simulink model "DualStreamSSR"  (R2023a)
(part 3 of 6)

  filter15 : aieBasic/AIE Class Kernel  KernelAllAttrs=|  PortNames={'sin1'; 'sin2'; 'cin'; 'sout1'; 'sout2'}  PortSerializedTypes={'{Q2{P{Tinput_stream{1{t{Scint16}}}}}}'; '{Q2{P{Tinput_stream{1{t{Scint16}}}}}}'; '{P{Tinput_stream{1{t{Scacc48_t}}}}}'; '{Q2{P{Toutput_stream{1{t{Scint16}}}}}}'; '{Q2{P{Toutput_stream{1{t{Scint16}}}}}}'}  PortWindowSizes={0.000000000000000000e+00; 0.000000000000000000e+00; 0.000000000000000000e+00; 0.000000000000000000e+00; 0.000000000000000000e+00}  PortWindowMargins={0.000000000000000000e+00; 0.000000000000000000e+00; 0.000000000000000000e+00; 0.000000000000000000e+00; 0.000000000000000000e+00}  PortSynchronicities={'auto', 'auto', 'auto', 'auto', 'auto'}  PortSignalSizes={0.000000000000000000e+00; 0.000000000000000000e+00; 0.000000000000000000e+00; 4.000000000000000000e+00; 4.000000000000000000e+00}  ClassTemplateSpecKind=implicit  ClassTemplateParamNames={'NSamples'; 'ShiftAcc'; 'DiscardSample'; 'SwapRead'}  ClassTemplateParamKinds={'nontype'; 'nontype'; 'nontype'; 'nontype'}  ClassTemplateParamTypes={'int'; 'int'; 'bool'; 'bool'}  ClassTemplateParamValues={'512', '15', '1', '0'}  ClassCtorParamNames={'taps'}  ClassCtorParamSerializedTypes={'{R{Q1{C{Scint16}4}}}'}  ClassCtorParamValues={'[342-439i 8773+2748i 102+525i -54+21i]'}  ClassIndex=1  ClassCtorIndex=1  ClassTabVisible=on  ClassTemplateParamsVisible=on  ClassCtorDeclVisible=on  ClassCtorParamsVisible=on  FunctionTabVisible=on  FunctionDecl=|  PortAttrs={ 'input', 'sin1', 'input_stream_cint16 * restrict', '', '', '', ''; 'input', 'sin2', 'input_stream_cint16 * restrict', '', '', '', ''; 'input', 'cin', 'input_stream< cacc48_t > *', '', '', '', ''; 'output', 'sout1', 'output_stream_cint16 * restrict', '', '', '', 'OUTPUT_SIZE/2'; 'output', 'sout2', 'output_stream_cint16 * restrict', '', '', '', 'OUTPUT_SIZE/2' }  PortAttrsEnables={'off', 'off', 'off', 'off', 'off', 'off', 'off';'off', 'off', 'off', 'off', 'off', 'off', 'off';'off', 'off', 'off', 'off', 'off', 'off', 'off';'off', 'off', 'off', 'off', 'off', 'off', 'on';'off', 'off', 'off', 'off', 'off', 'off', 'on'}  SampleTime=-1  ClassDeclTypeOptions=|  ClassDecl=|  ClassTemplateParams={ 'NSamples', 'int', 'BURST_LENGTH'; 'ShiftAcc', 'int', 'SHIFT_ACC'; 'DiscardSample', 'bool', 'TRUE'; 'SwapRead', 'bool', 'FALSE' }  ClassTemplateParamsEnables={'off', 'off', 'on';'off', 'off', 'on';'off', 'off', 'on';'off', 'off', 'on'}  ClassCtorDeclTypeOptions=C[1 1]@t50@FIR_MultiKernel_cin(cint16 const ( & taps ) [ 4 ])  ClassCtorDecl=FIR_MultiKernel_cin(cint16 const ( & taps ) [ 4 ])  ClassCtorParams={ 'taps', 'cint16 const ( &) [ 4 ]', 'phi_7' }  KernelHeaderFile=FirDoubleStream.h  KernelClassName=DoubleStream::FIR_MultiKernel_cin  KernelFunction=filter  KernelSourceFile=FirDoubleStream.cpp  KernelSearchPaths={'$SRC/aie_kernels'}  PreProcOptions={}  blockJsonConstraints="{\"type\":\"constraint\",\"constraintType\":\"location_kernel\",\"sid\":\"796\",\"lhs\":{\"type\":\"location\",\"templParam\":\"kernel\",\"args\":{\"type\":\"kernel\",\"name\":\"DualStreamSSR/SSR8/filter15\",\"sid\":\"796\"}},\"rhs\":{\"type\":\"tile\",\"args\":[{\"type\":\"evaluable\",\"expr\":\"23\",\"value\":23},{\"type\":\"evaluable\",\"expr\":\"1\",\"value\":1}]},\"equality\":true}"
      KernelAllAttrs=|
      | s[12;12;9;9;19;14;21;23;24;21;12;24;26;26;26;27;28;9;21;23;23;23;24;25;14;19;19;29]@FunctionNameDeclFileNamePortNamesPortTypesPortSerializedTypesPortDirectionsPortWindowSizeEnablesPortWindowMarginEnablesPortSynchronicityEnablesPortSignalSizeEnablesFunctionDeclFunctionTemplateSpecKindFunctionTemplateParamNamesFunctionTemplateParamKindsFunctionTemplateParamTypesFunctionTemplateParamValuesFunctionTemplateParamEnablesClassDeclClassTemplateSpecKindClassTemplateParamNamesClassTemplateParamKindsClassTemplateParamTypesClassTemplateParamValuesClassTemplateParamEnablesClassCtorDeclsClassCtorParamNamesClassCtorParamTypesClassCtorParamSerializedTypes[1 1]@C[28 1]@t6@filtert42@../../../aie/aie_kernels/FirDoubleStream.hC[5 1]@t4@sin1t4@sin2t3@cint5@sout1t5@sout2C[5 1]@t30@input_stream_cint16 * restrictt30@input_stream_cint16 * restrictt26@input_stream< cacc48_t > *t31@output_stream_cint16 * restrictt31@output_stream_cint16 * restrictC[5 1]@t37@{Q2{P{Tinput_stream{1{t{Scint16}}}}}}t37@{Q2{P{Tinput_stream{1{t{Scint16}}}}}}t35@{P{Tinput_stream{1{t{Scacc48_t}}}}}t38@{Q2{P{Toutput_stream{1{t{Scint16}}}}}}t38@{Q2{P{Toutput_stream{1{t{Scint16}}}}}}C[5 1]@t5@inputt5@inputt5@inputt6@outputt6@outputC[5 1]@l0@l0@l0@l0@l0@C[5 1]@l0@l0@l0@l0@l0@C[5 1]@l0@l0@l0@l0@l0@C[5 1]@l0@l0@l0@l1@l1@t321@namespace DoubleStream {
      | template < int NSamples, int ShiftAcc, bool DiscardSample, bool SwapRead > 
      | void FIR_MultiKernel_cin::
      | filter(input_stream_cint16 * restrict sin1, input_stream_cint16 * restrict sin2, input_stream< cacc48_t > * cin, output_stream_cint16 * restrict sout1, output_stream_cint16 * restrict sout2);
      | }t4@nonee[0 1]@e[0 1]@e[0 1]@e[0 1]@e[0 1]@t128@namespace DoubleStream {
      | template < int NSamples, int ShiftAcc, bool DiscardSample, bool SwapRead > class FIR_MultiKernel_cin;
      | }t8@implicitC[4 1]@t8@NSamplest8@ShiftAcct13@DiscardSamplet8@SwapReadC[4 1]@t7@nontypet7@nontypet7@nontypet7@nontypeC[4 1]@t3@intt3@intt4@boolt4@boolC[4 1]@nnnnC[4 1]@l1@l1@l1@l1@C[1 1]@t50@FIR_MultiKernel_cin(cint16 const ( & taps ) [ 4 ])C[1 1]@C[1 1]@t4@tapsC[1 1]@C[1 1]@t23@cint16 const ( &) [ 4 ]C[1 1]@C[1 1]@t20@{R{Q1{C{Scint16}4}}}
      FunctionDecl=|
      | namespace DoubleStream {
      | template < int NSamples, int ShiftAcc, bool DiscardSample, bool SwapRead > 
      | void FIR_MultiKernel_cin::
      | filter(input_stream_cint16 * restrict sin1, input_stream_cint16 * restrict sin2, input_stream< cacc48_t > * cin, output_stream_cint16 * restrict sout1, output_stream_cint16 * restrict sout2);
      | }
      ClassDeclTypeOptions=|
      | C[1 1]@t128@namespace DoubleStream {
      | template < int NSamples, int ShiftAcc, bool DiscardSample, bool SwapRead > class FIR_MultiKernel_cin;
      | }
      ClassDecl=|
      | namespace DoubleStream {
      | template < int NSamples, int ShiftAcc, bool DiscardSample, bool SwapRead > class FIR_MultiKernel_cin;
      | }
  filter16 : aieBasic/AIE Class Kernel  KernelAllAttrs=|  PortNames={'sin1'; 'sin2'; 'cout'}  PortSerializedTypes={'{Q2{P{Tinput_stream{1{t{Scint16}}}}}}'; '{Q2{P{Tinput_stream{1{t{Scint16}}}}}}'; '{P{Toutput_stream{1{t{Scacc48_t}}}}}'}  PortWindowSizes={0.000000000000000000e+00; 0.000000000000000000e+00; 0.000000000000000000e+00}  PortWindowMargins={0.000000000000000000e+00; 0.000000000000000000e+00; 0.000000000000000000e+00}  PortSynchronicities={'auto', 'auto', 'auto'}  PortSignalSizes={0.000000000000000000e+00; 0.000000000000000000e+00; 8.000000000000000000e+00}  ClassTemplateSpecKind=implicit  ClassTemplateParamNames={'NSamples'; 'ShiftAcc'; 'DiscardSample'; 'SwapRead'}  ClassTemplateParamKinds={'nontype'; 'nontype'; 'nontype'; 'nontype'}  ClassTemplateParamTypes={'int'; 'int'; 'bool'; 'bool'}  ClassTemplateParamValues={'512', '15', '1', '0'}  ClassCtorParamNames={'taps'}  ClassCtorParamSerializedTypes={'{R{Q1{C{Scint16}4}}}'}  ClassCtorParamValues={'[146-91i 4086+5221i 237-54i -83-21i]'}  ClassIndex=1  ClassCtorIndex=1  ClassTabVisible=on  ClassTemplateParamsVisible=on  ClassCtorDeclVisible=on  ClassCtorParamsVisible=on  FunctionTabVisible=on  FunctionDecl=|  PortAttrs={ 'input', 'sin1', 'input_stream_cint16 * restrict', '', '', '', ''; 'input', 'sin2', 'input_stream_cint16 * restrict', '', '', '', ''; 'output', 'cout', 'output_stream< cacc48_t > *', '', '', '', 'OUTPUT_SIZE' }  PortAttrsEnables={'off', 'off', 'off', 'off', 'off', 'off', 'off';'off', 'off', 'off', 'off', 'off', 'off', 'off';'off', 'off', 'off', 'off', 'off', 'off', 'on'}  SampleTime=-1  ClassDeclTypeOptions=|  ClassDecl=|  ClassTemplateParams={ 'NSamples', 'int', 'BURST_LENGTH'; 'ShiftAcc', 'int', 'SHIFT_ACC'; 'DiscardSample', 'bool', 'TRUE'; 'SwapRead', 'bool', 'FALSE' }  ClassTemplateParamsEnables={'off', 'off', 'on';'off', 'off', 'on';'off', 'off', 'on';'off', 'off', 'on'}  ClassCtorDeclTypeOptions=C[1 1]@t51@FIR_MultiKernel_cout(cint16 const ( & taps ) [ 4 ])  ClassCtorDecl=FIR_MultiKernel_cout(cint16 const ( & taps ) [ 4 ])  ClassCtorParams={ 'taps', 'cint16 const ( &) [ 4 ]', 'phi_6' }  KernelHeaderFile=FirDoubleStream.h  KernelClassName=DoubleStream::FIR_MultiKernel_cout  KernelFunction=filter  KernelSourceFile=FirDoubleStream.cpp  KernelSearchPaths={'$SRC/aie_kernels'}  PreProcOptions={}  blockJsonConstraints="{\"type\":\"constraint\",\"constraintType\":\"location_kernel\",\"sid\":\"797\",\"lhs\":{\"type\":\"location\",\"templParam\":\"kernel\",\"args\":{\"type\":\"kernel\",\"name\":\"DualStreamSSR/SSR8/filter16\",\"sid\":\"797\"}},\"rhs\":{\"type\":\"tile\",\"args\":[{\"type\":\"evaluable\",\"expr\":\"23\",\"value\":23},{\"type\":\"evaluable\",\"expr\":\"2\",\"value\":2}]},\"equality\":true}"
      KernelAllAttrs=|
      | s[12;12;9;9;19;14;21;23;24;21;12;24;26;26;26;27;28;9;21;23;23;23;24;25;14;19;19;29]@FunctionNameDeclFileNamePortNamesPortTypesPortSerializedTypesPortDirectionsPortWindowSizeEnablesPortWindowMarginEnablesPortSynchronicityEnablesPortSignalSizeEnablesFunctionDeclFunctionTemplateSpecKindFunctionTemplateParamNamesFunctionTemplateParamKindsFunctionTemplateParamTypesFunctionTemplateParamValuesFunctionTemplateParamEnablesClassDeclClassTemplateSpecKindClassTemplateParamNamesClassTemplateParamKindsClassTemplateParamTypesClassTemplateParamValuesClassTemplateParamEnablesClassCtorDeclsClassCtorParamNamesClassCtorParamTypesClassCtorParamSerializedTypes[1 1]@C[28 1]@t6@filtert42@../../../aie/aie_kernels/FirDoubleStream.hC[3 1]@t4@sin1t4@sin2t4@coutC[3 1]@t30@input_stream_cint16 * restrictt30@input_stream_cint16 * restrictt27@output_stream< cacc48_t > *C[3 1]@t37@{Q2{P{Tinput_stream{1{t{Scint16}}}}}}t37@{Q2{P{Tinput_stream{1{t{Scint16}}}}}}t36@{P{Toutput_stream{1{t{Scacc48_t}}}}}C[3 1]@t5@inputt5@inputt6@outputC[3 1]@l0@l0@l0@C[3 1]@l0@l0@l0@C[3 1]@l0@l0@l0@C[3 1]@l0@l0@l1@t246@namespace DoubleStream {
      | template < int NSamples, int ShiftAcc, bool DiscardSample, bool SwapRead > 
      | void FIR_MultiKernel_cout::
      | filter(input_stream_cint16 * restrict sin1, input_stream_cint16 * restrict sin2, output_stream< cacc48_t > * cout);
      | }t4@nonee[0 1]@e[0 1]@e[0 1]@e[0 1]@e[0 1]@t129@namespace DoubleStream {
      | template < int NSamples, int ShiftAcc, bool DiscardSample, bool SwapRead > class FIR_MultiKernel_cout;
      | }t8@implicitC[4 1]@t8@NSamplest8@ShiftAcct13@DiscardSamplet8@SwapReadC[4 1]@t7@nontypet7@nontypet7@nontypet7@nontypeC[4 1]@t3@intt3@intt4@boolt4@boolC[4 1]@nnnnC[4 1]@l1@l1@l1@l1@C[1 1]@t51@FIR_MultiKernel_cout(cint16 const ( & taps ) [ 4 ])C[1 1]@C[1 1]@t4@tapsC[1 1]@C[1 1]@t23@cint16 const ( &) [ 4 ]C[1 1]@C[1 1]@t20@{R{Q1{C{Scint16}4}}}
      FunctionDecl=|
      | namespace DoubleStream {
      | template < int NSamples, int ShiftAcc, bool DiscardSample, bool SwapRead > 
      | void FIR_MultiKernel_cout::
      | filter(input_stream_cint16 * restrict sin1, input_stream_cint16 * restrict sin2, output_stream< cacc48_t > * cout);
      | }
      ClassDeclTypeOptions=|
      | C[1 1]@t129@namespace DoubleStream {
      | template < int NSamples, int ShiftAcc, bool DiscardSample, bool SwapRead > class FIR_MultiKernel_cout;
      | }
      ClassDecl=|
      | namespace DoubleStream {
      | template < int NSamples, int ShiftAcc, bool DiscardSample, bool SwapRead > class FIR_MultiKernel_cout;
      | }
  filter17 : aieBasic/AIE Class Kernel  KernelAllAttrs=|  PortNames={'sin1'; 'sin2'; 'cin'; 'cout'}  PortSerializedTypes={'{Q2{P{Tinput_stream{1{t{Scint16}}}}}}'; '{Q2{P{Tinput_stream{1{t{Scint16}}}}}}'; '{P{Tinput_stream{1{t{Scacc48_t}}}}}'; '{P{Toutput_stream{1{t{Scacc48_t}}}}}'}  PortWindowSizes={0.000000000000000000e+00; 0.000000000000000000e+00; 0.000000000000000000e+00; 0.000000000000000000e+00}  PortWindowMargins={0.000000000000000000e+00; 0.000000000000000000e+00; 0.000000000000000000e+00; 0.000000000000000000e+00}  PortSynchronicities={'auto', 'auto', 'auto', 'auto'}  PortSignalSizes={0.000000000000000000e+00; 0.000000000000000000e+00; 0.000000000000000000e+00; 8.000000000000000000e+00}  ClassTemplateSpecKind=implicit  ClassTemplateParamNames={'NSamples'; 'ShiftAcc'; 'DiscardSample'; 'SwapRead'}  ClassTemplateParamKinds={'nontype'; 'nontype'; 'nontype'; 'nontype'}  ClassTemplateParamTypes={'int'; 'int'; 'bool'; 'bool'}  ClassTemplateParamValues={'512', '15', '1', '0'}  ClassCtorParamNames={'taps'}  ClassCtorParamSerializedTypes={'{R{Q1{C{Scint16}4}}}'}  ClassCtorParamValues={'[342-439i 8773+2748i 102+525i -54+21i]'}  ClassIndex=1  ClassCtorIndex=1  ClassTabVisible=on  ClassTemplateParamsVisible=on  ClassCtorDeclVisible=on  ClassCtorParamsVisible=on  FunctionTabVisible=on  FunctionDecl=|  PortAttrs={ 'input', 'sin1', 'input_stream_cint16 * restrict', '', '', '', ''; 'input', 'sin2', 'input_stream_cint16 * restrict', '', '', '', ''; 'input', 'cin', 'input_stream< cacc48_t > *', '', '', '', ''; 'output', 'cout', 'output_stream< cacc48_t > *', '', '', '', 'OUTPUT_SIZE' }  PortAttrsEnables={'off', 'off', 'off', 'off', 'off', 'off', 'off';'off', 'off', 'off', 'off', 'off', 'off', 'off';'off', 'off', 'off', 'off', 'off', 'off', 'off';'off', 'off', 'off', 'off', 'off', 'off', 'on'}  SampleTime=-1  ClassDeclTypeOptions=|  ClassDecl=|  ClassTemplateParams={ 'NSamples', 'int', 'BURST_LENGTH'; 'ShiftAcc', 'int', 'SHIFT_ACC'; 'DiscardSample', 'bool', 'TRUE'; 'SwapRead', 'bool', 'FALSE' }  ClassTemplateParamsEnables={'off', 'off', 'on';'off', 'off', 'on';'off', 'off', 'on';'off', 'off', 'on'}  ClassCtorDeclTypeOptions=C[1 1]@t54@FIR_MultiKernel_cincout(cint16 const ( & taps ) [ 4 ])  ClassCtorDecl=FIR_MultiKernel_cincout(cint16 const ( & taps ) [ 4 ])  ClassCtorParams={ 'taps', 'cint16 const ( &) [ 4 ]', 'phi_7' }  KernelHeaderFile=FirDoubleStream.h  KernelClassName=DoubleStream::FIR_MultiKernel_cincout  KernelFunction=filter  KernelSourceFile=FirDoubleStream.cpp  KernelSearchPaths={'$SRC/aie_kernels'}  PreProcOptions={}  blockJsonConstraints="{\"type\":\"constraint\",\"constraintType\":\"location_kernel\",\"sid\":\"798\",\"lhs\":{\"type\":\"location\",\"templParam\":\"kernel\",\"args\":{\"type\":\"kernel\",\"name\":\"DualStreamSSR/SSR8/filter17\",\"sid\":\"798\"}},\"rhs\":{\"type\":\"tile\",\"args\":[{\"type\":\"evaluable\",\"expr\":\"24\",\"value\":24},{\"type\":\"evaluable\",\"expr\":\"2\",\"value\":2}]},\"equality\":true}"
      KernelAllAttrs=|
      | s[12;12;9;9;19;14;21;23;24;21;12;24;26;26;26;27;28;9;21;23;23;23;24;25;14;19;19;29]@FunctionNameDeclFileNamePortNamesPortTypesPortSerializedTypesPortDirectionsPortWindowSizeEnablesPortWindowMarginEnablesPortSynchronicityEnablesPortSignalSizeEnablesFunctionDeclFunctionTemplateSpecKindFunctionTemplateParamNamesFunctionTemplateParamKindsFunctionTemplateParamTypesFunctionTemplateParamValuesFunctionTemplateParamEnablesClassDeclClassTemplateSpecKindClassTemplateParamNamesClassTemplateParamKindsClassTemplateParamTypesClassTemplateParamValuesClassTemplateParamEnablesClassCtorDeclsClassCtorParamNamesClassCtorParamTypesClassCtorParamSerializedTypes[1 1]@C[28 1]@t6@filtert42@../../../aie/aie_kernels/FirDoubleStream.hC[4 1]@t4@sin1t4@sin2t3@cint4@coutC[4 1]@t30@input_stream_cint16 * restrictt30@input_stream_cint16 * restrictt26@input_stream< cacc48_t > *t27@output_stream< cacc48_t > *C[4 1]@t37@{Q2{P{Tinput_stream{1{t{Scint16}}}}}}t37@{Q2{P{Tinput_stream{1{t{Scint16}}}}}}t35@{P{Tinput_stream{1{t{Scacc48_t}}}}}t36@{P{Toutput_stream{1{t{Scacc48_t}}}}}C[4 1]@t5@inputt5@inputt5@inputt6@outputC[4 1]@l0@l0@l0@l0@C[4 1]@l0@l0@l0@l0@C[4 1]@l0@l0@l0@l0@C[4 1]@l0@l0@l0@l1@t281@namespace DoubleStream {
      | template < int NSamples, int ShiftAcc, bool DiscardSample, bool SwapRead > 
      | void FIR_MultiKernel_cincout::
      | filter(input_stream_cint16 * restrict sin1, input_stream_cint16 * restrict sin2, input_stream< cacc48_t > * cin, output_stream< cacc48_t > * cout);
      | }t4@nonee[0 1]@e[0 1]@e[0 1]@e[0 1]@e[0 1]@t132@namespace DoubleStream {
      | template < int NSamples, int ShiftAcc, bool DiscardSample, bool SwapRead > class FIR_MultiKernel_cincout;
      | }t8@implicitC[4 1]@t8@NSamplest8@ShiftAcct13@DiscardSamplet8@SwapReadC[4 1]@t7@nontypet7@nontypet7@nontypet7@nontypeC[4 1]@t3@intt3@intt4@boolt4@boolC[4 1]@nnnnC[4 1]@l1@l1@l1@l1@C[1 1]@t54@FIR_MultiKernel_cincout(cint16 const ( & taps ) [ 4 ])C[1 1]@C[1 1]@t4@tapsC[1 1]@C[1 1]@t23@cint16 const ( &) [ 4 ]C[1 1]@C[1 1]@t20@{R{Q1{C{Scint16}4}}}
      FunctionDecl=|
      | namespace DoubleStream {
      | template < int NSamples, int ShiftAcc, bool DiscardSample, bool SwapRead > 
      | void FIR_MultiKernel_cincout::
      | filter(input_stream_cint16 * restrict sin1, input_stream_cint16 * restrict sin2, input_stream< cacc48_t > * cin, output_stream< cacc48_t > * cout);
      | }
      ClassDeclTypeOptions=|
      | C[1 1]@t132@namespace DoubleStream {
      | template < int NSamples, int ShiftAcc, bool DiscardSample, bool SwapRead > class FIR_MultiKernel_cincout;
      | }
      ClassDecl=|
      | namespace DoubleStream {
      | template < int NSamples, int ShiftAcc, bool DiscardSample, bool SwapRead > class FIR_MultiKernel_cincout;
      | }
  filter18 : aieBasic/AIE Class Kernel  KernelAllAttrs=|  PortNames={'sin1'; 'sin2'; 'cin'; 'cout'}  PortSerializedTypes={'{Q2{P{Tinput_stream{1{t{Scint16}}}}}}'; '{Q2{P{Tinput_stream{1{t{Scint16}}}}}}'; '{P{Tinput_stream{1{t{Scacc48_t}}}}}'; '{P{Toutput_stream{1{t{Scacc48_t}}}}}'}  PortWindowSizes={0.000000000000000000e+00; 0.000000000000000000e+00; 0.000000000000000000e+00; 0.000000000000000000e+00}  PortWindowMargins={0.000000000000000000e+00; 0.000000000000000000e+00; 0.000000000000000000e+00; 0.000000000000000000e+00}  PortSynchronicities={'auto', 'auto', 'auto', 'auto'}  PortSignalSizes={0.000000000000000000e+00; 0.000000000000000000e+00; 0.000000000000000000e+00; 8.000000000000000000e+00}  ClassTemplateSpecKind=implicit  ClassTemplateParamNames={'NSamples'; 'ShiftAcc'; 'DiscardSample'; 'SwapRead'}  ClassTemplateParamKinds={'nontype'; 'nontype'; 'nontype'; 'nontype'}  ClassTemplateParamTypes={'int'; 'int'; 'bool'; 'bool'}  ClassTemplateParamValues={'512', '15', '1', '0'}  ClassCtorParamNames={'taps'}  ClassCtorParamSerializedTypes={'{R{Q1{C{Scint16}4}}}'}  ClassCtorParamValues={'[342-439i 8773+2748i 102+525i -54+21i]'}  ClassIndex=1  ClassCtorIndex=1  ClassTabVisible=on  ClassTemplateParamsVisible=on  ClassCtorDeclVisible=on  ClassCtorParamsVisible=on  FunctionTabVisible=on  FunctionDecl=|  PortAttrs={ 'input', 'sin1', 'input_stream_cint16 * restrict', '', '', '', ''; 'input', 'sin2', 'input_stream_cint16 * restrict', '', '', '', ''; 'input', 'cin', 'input_stream< cacc48_t > *', '', '', '', ''; 'output', 'cout', 'output_stream< cacc48_t > *', '', '', '', 'OUTPUT_SIZE' }  PortAttrsEnables={'off', 'off', 'off', 'off', 'off', 'off', 'off';'off', 'off', 'off', 'off', 'off', 'off', 'off';'off', 'off', 'off', 'off', 'off', 'off', 'off';'off', 'off', 'off', 'off', 'off', 'off', 'on'}  SampleTime=-1  ClassDeclTypeOptions=|  ClassDecl=|  ClassTemplateParams={ 'NSamples', 'int', 'BURST_LENGTH'; 'ShiftAcc', 'int', 'SHIFT_ACC'; 'DiscardSample', 'bool', 'TRUE'; 'SwapRead', 'bool', 'FALSE' }  ClassTemplateParamsEnables={'off', 'off', 'on';'off', 'off', 'on';'off', 'off', 'on';'off', 'off', 'on'}  ClassCtorDeclTypeOptions=C[1 1]@t54@FIR_MultiKernel_cincout(cint16 const ( & taps ) [ 4 ])  ClassCtorDecl=FIR_MultiKernel_cincout(cint16 const ( & taps ) [ 4 ])  ClassCtorParams={ 'taps', 'cint16 const ( &) [ 4 ]', 'phi_7' }  KernelHeaderFile=FirDoubleStream.h  KernelClassName=DoubleStream::FIR_MultiKernel_cincout  KernelFunction=filter  KernelSourceFile=FirDoubleStream.cpp  KernelSearchPaths={'$SRC/aie_kernels'}  PreProcOptions={}  blockJsonConstraints="{\"type\":\"constraint\",\"constraintType\":\"location_kernel\",\"sid\":\"799\",\"lhs\":{\"type\":\"location\",\"templParam\":\"kernel\",\"args\":{\"type\":\"kernel\",\"name\":\"DualStreamSSR/SSR8/filter18\",\"sid\":\"799\"}},\"rhs\":{\"type\":\"tile\",\"args\":[{\"type\":\"evaluable\",\"expr\":\"25\",\"value\":25},{\"type\":\"evaluable\",\"expr\":\"3\",\"value\":3}]},\"equality\":true}"
      KernelAllAttrs=|
      | s[12;12;9;9;19;14;21;23;24;21;12;24;26;26;26;27;28;9;21;23;23;23;24;25;14;19;19;29]@FunctionNameDeclFileNamePortNamesPortTypesPortSerializedTypesPortDirectionsPortWindowSizeEnablesPortWindowMarginEnablesPortSynchronicityEnablesPortSignalSizeEnablesFunctionDeclFunctionTemplateSpecKindFunctionTemplateParamNamesFunctionTemplateParamKindsFunctionTemplateParamTypesFunctionTemplateParamValuesFunctionTemplateParamEnablesClassDeclClassTemplateSpecKindClassTemplateParamNamesClassTemplateParamKindsClassTemplateParamTypesClassTemplateParamValuesClassTemplateParamEnablesClassCtorDeclsClassCtorParamNamesClassCtorParamTypesClassCtorParamSerializedTypes[1 1]@C[28 1]@t6@filtert42@../../../aie/aie_kernels/FirDoubleStream.hC[4 1]@t4@sin1t4@sin2t3@cint4@coutC[4 1]@t30@input_stream_cint16 * restrictt30@input_stream_cint16 * restrictt26@input_stream< cacc48_t > *t27@output_stream< cacc48_t > *C[4 1]@t37@{Q2{P{Tinput_stream{1{t{Scint16}}}}}}t37@{Q2{P{Tinput_stream{1{t{Scint16}}}}}}t35@{P{Tinput_stream{1{t{Scacc48_t}}}}}t36@{P{Toutput_stream{1{t{Scacc48_t}}}}}C[4 1]@t5@inputt5@inputt5@inputt6@outputC[4 1]@l0@l0@l0@l0@C[4 1]@l0@l0@l0@l0@C[4 1]@l0@l0@l0@l0@C[4 1]@l0@l0@l0@l1@t281@namespace DoubleStream {
      | template < int NSamples, int ShiftAcc, bool DiscardSample, bool SwapRead > 
      | void FIR_MultiKernel_cincout::
      | filter(input_stream_cint16 * restrict sin1, input_stream_cint16 * restrict sin2, input_stream< cacc48_t > * cin, output_stream< cacc48_t > * cout);
      | }t4@nonee[0 1]@e[0 1]@e[0 1]@e[0 1]@e[0 1]@t132@namespace DoubleStream {
      | template < int NSamples, int ShiftAcc, bool DiscardSample, bool SwapRead > class FIR_MultiKernel_cincout;
      | }t8@implicitC[4 1]@t8@NSamplest8@ShiftAcct13@DiscardSamplet8@SwapReadC[4 1]@t7@nontypet7@nontypet7@nontypet7@nontypeC[4 1]@t3@intt3@intt4@boolt4@boolC[4 1]@nnnnC[4 1]@l1@l1@l1@l1@C[1 1]@t54@FIR_MultiKernel_cincout(cint16 const ( & taps ) [ 4 ])C[1 1]@C[1 1]@t4@tapsC[1 1]@C[1 1]@t23@cint16 const ( &) [ 4 ]C[1 1]@C[1 1]@t20@{R{Q1{C{Scint16}4}}}
      FunctionDecl=|
      | namespace DoubleStream {
      | template < int NSamples, int ShiftAcc, bool DiscardSample, bool SwapRead > 
      | void FIR_MultiKernel_cincout::
      | filter(input_stream_cint16 * restrict sin1, input_stream_cint16 * restrict sin2, input_stream< cacc48_t > * cin, output_stream< cacc48_t > * cout);
      | }
      ClassDeclTypeOptions=|
      | C[1 1]@t132@namespace DoubleStream {
      | template < int NSamples, int ShiftAcc, bool DiscardSample, bool SwapRead > class FIR_MultiKernel_cincout;
      | }
      ClassDecl=|
      | namespace DoubleStream {
      | template < int NSamples, int ShiftAcc, bool DiscardSample, bool SwapRead > class FIR_MultiKernel_cincout;
      | }
  filter19 : aieBasic/AIE Class Kernel  KernelAllAttrs=|  PortNames={'sin1'; 'sin2'; 'cin'; 'cout'}  PortSerializedTypes={'{Q2{P{Tinput_stream{1{t{Scint16}}}}}}'; '{Q2{P{Tinput_stream{1{t{Scint16}}}}}}'; '{P{Tinput_stream{1{t{Scacc48_t}}}}}'; '{P{Toutput_stream{1{t{Scacc48_t}}}}}'}  PortWindowSizes={0.000000000000000000e+00; 0.000000000000000000e+00; 0.000000000000000000e+00; 0.000000000000000000e+00}  PortWindowMargins={0.000000000000000000e+00; 0.000000000000000000e+00; 0.000000000000000000e+00; 0.000000000000000000e+00}  PortSynchronicities={'auto', 'auto', 'auto', 'auto'}  PortSignalSizes={0.000000000000000000e+00; 0.000000000000000000e+00; 0.000000000000000000e+00; 8.000000000000000000e+00}  ClassTemplateSpecKind=implicit  ClassTemplateParamNames={'NSamples'; 'ShiftAcc'; 'DiscardSample'; 'SwapRead'}  ClassTemplateParamKinds={'nontype'; 'nontype'; 'nontype'; 'nontype'}  ClassTemplateParamTypes={'int'; 'int'; 'bool'; 'bool'}  ClassTemplateParamValues={'512', '15', '0', '0'}  ClassCtorParamNames={'taps'}  ClassCtorParamSerializedTypes={'{R{Q1{C{Scint16}4}}}'}  ClassCtorParamValues={'[-54-21i 102-525i 8773-2748i 342+439i]'}  ClassIndex=1  ClassCtorIndex=1  ClassTabVisible=on  ClassTemplateParamsVisible=on  ClassCtorDeclVisible=on  ClassCtorParamsVisible=on  FunctionTabVisible=on  FunctionDecl=|  PortAttrs={ 'input', 'sin1', 'input_stream_cint16 * restrict', '', '', '', ''; 'input', 'sin2', 'input_stream_cint16 * restrict', '', '', '', ''; 'input', 'cin', 'input_stream< cacc48_t > *', '', '', '', ''; 'output', 'cout', 'output_stream< cacc48_t > *', '', '', '', 'OUTPUT_SIZE' }  PortAttrsEnables={'off', 'off', 'off', 'off', 'off', 'off', 'off';'off', 'off', 'off', 'off', 'off', 'off', 'off';'off', 'off', 'off', 'off', 'off', 'off', 'off';'off', 'off', 'off', 'off', 'off', 'off', 'on'}  SampleTime=-1  ClassDeclTypeOptions=|  ClassDecl=|  ClassTemplateParams={ 'NSamples', 'int', 'BURST_LENGTH'; 'ShiftAcc', 'int', 'SHIFT_ACC'; 'DiscardSample', 'bool', 'FALSE'; 'SwapRead', 'bool', 'FALSE' }  ClassTemplateParamsEnables={'off', 'off', 'on';'off', 'off', 'on';'off', 'off', 'on';'off', 'off', 'on'}  ClassCtorDeclTypeOptions=C[1 1]@t54@FIR_MultiKernel_cincout(cint16 const ( & taps ) [ 4 ])  ClassCtorDecl=FIR_MultiKernel_cincout(cint16 const ( & taps ) [ 4 ])  ClassCtorParams={ 'taps', 'cint16 const ( &) [ 4 ]', 'phi_0' }  KernelHeaderFile=FirDoubleStream.h  KernelClassName=DoubleStream::FIR_MultiKernel_cincout  KernelFunction=filter  KernelSourceFile=FirDoubleStream.cpp  KernelSearchPaths={'$SRC/aie_kernels'}  PreProcOptions={}  blockJsonConstraints="{\"type\":\"constraint\",\"constraintType\":\"location_kernel\",\"sid\":\"800\",\"lhs\":{\"type\":\"location\",\"templParam\":\"kernel\",\"args\":{\"type\":\"kernel\",\"name\":\"DualStreamSSR/SSR8/filter19\",\"sid\":\"800\"}},\"rhs\":{\"type\":\"tile\",\"args\":[{\"type\":\"evaluable\",\"expr\":\"26\",\"value\":26},{\"type\":\"evaluable\",\"expr\":\"3\",\"value\":3}]},\"equality\":true}"
      KernelAllAttrs=|
      | s[12;12;9;9;19;14;21;23;24;21;12;24;26;26;26;27;28;9;21;23;23;23;24;25;14;19;19;29]@FunctionNameDeclFileNamePortNamesPortTypesPortSerializedTypesPortDirectionsPortWindowSizeEnablesPortWindowMarginEnablesPortSynchronicityEnablesPortSignalSizeEnablesFunctionDeclFunctionTemplateSpecKindFunctionTemplateParamNamesFunctionTemplateParamKindsFunctionTemplateParamTypesFunctionTemplateParamValuesFunctionTemplateParamEnablesClassDeclClassTemplateSpecKindClassTemplateParamNamesClassTemplateParamKindsClassTemplateParamTypesClassTemplateParamValuesClassTemplateParamEnablesClassCtorDeclsClassCtorParamNamesClassCtorParamTypesClassCtorParamSerializedTypes[1 1]@C[28 1]@t6@filtert42@../../../aie/aie_kernels/FirDoubleStream.hC[4 1]@t4@sin1t4@sin2t3@cint4@coutC[4 1]@t30@input_stream_cint16 * restrictt30@input_stream_cint16 * restrictt26@input_stream< cacc48_t > *t27@output_stream< cacc48_t > *C[4 1]@t37@{Q2{P{Tinput_stream{1{t{Scint16}}}}}}t37@{Q2{P{Tinput_stream{1{t{Scint16}}}}}}t35@{P{Tinput_stream{1{t{Scacc48_t}}}}}t36@{P{Toutput_stream{1{t{Scacc48_t}}}}}C[4 1]@t5@inputt5@inputt5@inputt6@outputC[4 1]@l0@l0@l0@l0@C[4 1]@l0@l0@l0@l0@C[4 1]@l0@l0@l0@l0@C[4 1]@l0@l0@l0@l1@t281@namespace DoubleStream {
      | template < int NSamples, int ShiftAcc, bool DiscardSample, bool SwapRead > 
      | void FIR_MultiKernel_cincout::
      | filter(input_stream_cint16 * restrict sin1, input_stream_cint16 * restrict sin2, input_stream< cacc48_t > * cin, output_stream< cacc48_t > * cout);
      | }t4@nonee[0 1]@e[0 1]@e[0 1]@e[0 1]@e[0 1]@t132@namespace DoubleStream {
      | template < int NSamples, int ShiftAcc, bool DiscardSample, bool SwapRead > class FIR_MultiKernel_cincout;
      | }t8@implicitC[4 1]@t8@NSamplest8@ShiftAcct13@DiscardSamplet8@SwapReadC[4 1]@t7@nontypet7@nontypet7@nontypet7@nontypeC[4 1]@t3@intt3@intt4@boolt4@boolC[4 1]@nnnnC[4 1]@l1@l1@l1@l1@C[1 1]@t54@FIR_MultiKernel_cincout(cint16 const ( & taps ) [ 4 ])C[1 1]@C[1 1]@t4@tapsC[1 1]@C[1 1]@t23@cint16 const ( &) [ 4 ]C[1 1]@C[1 1]@t20@{R{Q1{C{Scint16}4}}}
      FunctionDecl=|
      | namespace DoubleStream {
      | template < int NSamples, int ShiftAcc, bool DiscardSample, bool SwapRead > 
      | void FIR_MultiKernel_cincout::
      | filter(input_stream_cint16 * restrict sin1, input_stream_cint16 * restrict sin2, input_stream< cacc48_t > * cin, output_stream< cacc48_t > * cout);
      | }
      ClassDeclTypeOptions=|
      | C[1 1]@t132@namespace DoubleStream {
      | template < int NSamples, int ShiftAcc, bool DiscardSample, bool SwapRead > class FIR_MultiKernel_cincout;
      | }
      ClassDecl=|
      | namespace DoubleStream {
      | template < int NSamples, int ShiftAcc, bool DiscardSample, bool SwapRead > class FIR_MultiKernel_cincout;
      | }
  filter2 : aieBasic/AIE Class Kernel  KernelAllAttrs=|  PortNames={'sin1'; 'sin2'; 'cin'; 'cout'}  PortSerializedTypes={'{Q2{P{Tinput_stream{1{t{Scint16}}}}}}'; '{Q2{P{Tinput_stream{1{t{Scint16}}}}}}'; '{P{Tinput_stream{1{t{Scacc48_t}}}}}'; '{P{Toutput_stream{1{t{Scacc48_t}}}}}'}  PortWindowSizes={0.000000000000000000e+00; 0.000000000000000000e+00; 0.000000000000000000e+00; 0.000000000000000000e+00}  PortWindowMargins={0.000000000000000000e+00; 0.000000000000000000e+00; 0.000000000000000000e+00; 0.000000000000000000e+00}  PortSynchronicities={'auto', 'auto', 'auto', 'auto'}  PortSignalSizes={0.000000000000000000e+00; 0.000000000000000000e+00; 0.000000000000000000e+00; 8.000000000000000000e+00}  ClassTemplateSpecKind=implicit  ClassTemplateParamNames={'NSamples'; 'ShiftAcc'; 'DiscardSample'; 'SwapRead'}  ClassTemplateParamKinds={'nontype'; 'nontype'; 'nontype'; 'nontype'}  ClassTemplateParamTypes={'int'; 'int'; 'bool'; 'bool'}  ClassTemplateParamValues={'512', '15', '0', '0'}  ClassCtorParamNames={'taps'}  ClassCtorParamSerializedTypes={'{R{Q1{C{Scint16}4}}}'}  ClassCtorParamValues={'[-21+26i 1183+239i 248-2878i -160+111i]'}  ClassIndex=1  ClassCtorIndex=1  ClassTabVisible=on  ClassTemplateParamsVisible=on  ClassCtorDeclVisible=on  ClassCtorParamsVisible=on  FunctionTabVisible=on  FunctionDecl=|  PortAttrs={ 'input', 'sin1', 'input_stream_cint16 * restrict', '', '', '', ''; 'input', 'sin2', 'input_stream_cint16 * restrict', '', '', '', ''; 'input', 'cin', 'input_stream< cacc48_t > *', '', '', '', ''; 'output', 'cout', 'output_stream< cacc48_t > *', '', '', '', 'OUTPUT_SIZE' }  PortAttrsEnables={'off', 'off', 'off', 'off', 'off', 'off', 'off';'off', 'off', 'off', 'off', 'off', 'off', 'off';'off', 'off', 'off', 'off', 'off', 'off', 'off';'off', 'off', 'off', 'off', 'off', 'off', 'on'}  SampleTime=-1  ClassDeclTypeOptions=|  ClassDecl=|  ClassTemplateParams={ 'NSamples', 'int', 'BURST_LENGTH'; 'ShiftAcc', 'int', 'SHIFT_ACC'; 'DiscardSample', 'bool', 'FALSE'; 'SwapRead', 'bool', 'FALSE' }  ClassTemplateParamsEnables={'off', 'off', 'on';'off', 'off', 'on';'off', 'off', 'on';'off', 'off', 'on'}  ClassCtorDeclTypeOptions=C[1 1]@t54@FIR_MultiKernel_cincout(cint16 const ( & taps ) [ 4 ])  ClassCtorDecl=FIR_MultiKernel_cincout(cint16 const ( & taps ) [ 4 ])  ClassCtorParams={ 'taps', 'cint16 const ( &) [ 4 ]', 'phi_2' }  KernelHeaderFile=FirDoubleStream.h  KernelClassName=DoubleStream::FIR_MultiKernel_cincout  KernelFunction=filter  KernelSourceFile=FirDoubleStream.cpp  KernelSearchPaths={'$SRC/aie_kernels'}  PreProcOptions={}  blockJsonConstraints="{\"type\":\"constraint\",\"constraintType\":\"location_kernel\",\"sid\":\"801\",\"lhs\":{\"type\":\"location\",\"templParam\":\"kernel\",\"args\":{\"type\":\"kernel\",\"name\":\"DualStreamSSR/SSR8/filter2\",\"sid\":\"801\"}},\"rhs\":{\"type\":\"tile\",\"args\":[{\"type\":\"evaluable\",\"expr\":\"25\",\"value\":25},{\"type\":\"evaluable\",\"expr\":\"0\",\"value\":0}]},\"equality\":true}"
      KernelAllAttrs=|
      | s[12;12;9;9;19;14;21;23;24;21;12;24;26;26;26;27;28;9;21;23;23;23;24;25;14;19;19;29]@FunctionNameDeclFileNamePortNamesPortTypesPortSerializedTypesPortDirectionsPortWindowSizeEnablesPortWindowMarginEnablesPortSynchronicityEnablesPortSignalSizeEnablesFunctionDeclFunctionTemplateSpecKindFunctionTemplateParamNamesFunctionTemplateParamKindsFunctionTemplateParamTypesFunctionTemplateParamValuesFunctionTemplateParamEnablesClassDeclClassTemplateSpecKindClassTemplateParamNamesClassTemplateParamKindsClassTemplateParamTypesClassTemplateParamValuesClassTemplateParamEnablesClassCtorDeclsClassCtorParamNamesClassCtorParamTypesClassCtorParamSerializedTypes[1 1]@C[28 1]@t6@filtert42@../../../aie/aie_kernels/FirDoubleStream.hC[4 1]@t4@sin1t4@sin2t3@cint4@coutC[4 1]@t30@input_stream_cint16 * restrictt30@input_stream_cint16 * restrictt26@input_stream< cacc48_t > *t27@output_stream< cacc48_t > *C[4 1]@t37@{Q2{P{Tinput_stream{1{t{Scint16}}}}}}t37@{Q2{P{Tinput_stream{1{t{Scint16}}}}}}t35@{P{Tinput_stream{1{t{Scacc48_t}}}}}t36@{P{Toutput_stream{1{t{Scacc48_t}}}}}C[4 1]@t5@inputt5@inputt5@inputt6@outputC[4 1]@l0@l0@l0@l0@C[4 1]@l0@l0@l0@l0@C[4 1]@l0@l0@l0@l0@C[4 1]@l0@l0@l0@l1@t281@namespace DoubleStream {
      | template < int NSamples, int ShiftAcc, bool DiscardSample, bool SwapRead > 
      | void FIR_MultiKernel_cincout::
      | filter(input_stream_cint16 * restrict sin1, input_stream_cint16 * restrict sin2, input_stream< cacc48_t > * cin, output_stream< cacc48_t > * cout);
      | }t4@nonee[0 1]@e[0 1]@e[0 1]@e[0 1]@e[0 1]@t132@namespace DoubleStream {
      | template < int NSamples, int ShiftAcc, bool DiscardSample, bool SwapRead > class FIR_MultiKernel_cincout;
      | }t8@implicitC[4 1]@t8@NSamplest8@ShiftAcct13@DiscardSamplet8@SwapReadC[4 1]@t7@nontypet7@nontypet7@nontypet7@nontypeC[4 1]@t3@intt3@intt4@boolt4@boolC[4 1]@nnnnC[4 1]@l1@l1@l1@l1@C[1 1]@t54@FIR_MultiKernel_cincout(cint16 const ( & taps ) [ 4 ])C[1 1]@C[1 1]@t4@tapsC[1 1]@C[1 1]@t23@cint16 const ( &) [ 4 ]C[1 1]@C[1 1]@t20@{R{Q1{C{Scint16}4}}}
      FunctionDecl=|
      | namespace DoubleStream {
      | template < int NSamples, int ShiftAcc, bool DiscardSample, bool SwapRead > 
      | void FIR_MultiKernel_cincout::
      | filter(input_stream_cint16 * restrict sin1, input_stream_cint16 * restrict sin2, input_stream< cacc48_t > * cin, output_stream< cacc48_t > * cout);
      | }
      ClassDeclTypeOptions=|
      | C[1 1]@t132@namespace DoubleStream {
      | template < int NSamples, int ShiftAcc, bool DiscardSample, bool SwapRead > class FIR_MultiKernel_cincout;
      | }
      ClassDecl=|
      | namespace DoubleStream {
      | template < int NSamples, int ShiftAcc, bool DiscardSample, bool SwapRead > class FIR_MultiKernel_cincout;
      | }
  filter20 : aieBasic/AIE Class Kernel  KernelAllAttrs=|  PortNames={'sin1'; 'sin2'; 'cin'; 'cout'}  PortSerializedTypes={'{Q2{P{Tinput_stream{1{t{Scint16}}}}}}'; '{Q2{P{Tinput_stream{1{t{Scint16}}}}}}'; '{P{Tinput_stream{1{t{Scacc48_t}}}}}'; '{P{Toutput_stream{1{t{Scacc48_t}}}}}'}  PortWindowSizes={0.000000000000000000e+00; 0.000000000000000000e+00; 0.000000000000000000e+00; 0.000000000000000000e+00}  PortWindowMargins={0.000000000000000000e+00; 0.000000000000000000e+00; 0.000000000000000000e+00; 0.000000000000000000e+00}  PortSynchronicities={'auto', 'auto', 'auto', 'auto'}  PortSignalSizes={0.000000000000000000e+00; 0.000000000000000000e+00; 0.000000000000000000e+00; 8.000000000000000000e+00}  ClassTemplateSpecKind=implicit  ClassTemplateParamNames={'NSamples'; 'ShiftAcc'; 'DiscardSample'; 'SwapRead'}  ClassTemplateParamKinds={'nontype'; 'nontype'; 'nontype'; 'nontype'}  ClassTemplateParamTypes={'int'; 'int'; 'bool'; 'bool'}  ClassTemplateParamValues={'512', '15', '0', '0'}  ClassCtorParamNames={'taps'}  ClassCtorParamSerializedTypes={'{R{Q1{C{Scint16}4}}}'}  ClassCtorParamValues={'[-83+21i 237+54i 4086-5221i 146+91i]'}  ClassIndex=1  ClassCtorIndex=1  ClassTabVisible=on  ClassTemplateParamsVisible=on  ClassCtorDeclVisible=on  ClassCtorParamsVisible=on  FunctionTabVisible=on  FunctionDecl=|  PortAttrs={ 'input', 'sin1', 'input_stream_cint16 * restrict', '', '', '', ''; 'input', 'sin2', 'input_stream_cint16 * restrict', '', '', '', ''; 'input', 'cin', 'input_stream< cacc48_t > *', '', '', '', ''; 'output', 'cout', 'output_stream< cacc48_t > *', '', '', '', 'OUTPUT_SIZE' }  PortAttrsEnables={'off', 'off', 'off', 'off', 'off', 'off', 'off';'off', 'off', 'off', 'off', 'off', 'off', 'off';'off', 'off', 'off', 'off', 'off', 'off', 'off';'off', 'off', 'off', 'off', 'off', 'off', 'on'}  SampleTime=-1  ClassDeclTypeOptions=|  ClassDecl=|  ClassTemplateParams={ 'NSamples', 'int', 'BURST_LENGTH'; 'ShiftAcc', 'int', 'SHIFT_ACC'; 'DiscardSample', 'bool', 'FALSE'; 'SwapRead', 'bool', 'FALSE' }  ClassTemplateParamsEnables={'off', 'off', 'on';'off', 'off', 'on';'off', 'off', 'on';'off', 'off', 'on'}  ClassCtorDeclTypeOptions=C[1 1]@t54@FIR_MultiKernel_cincout(cint16 const ( & taps ) [ 4 ])  ClassCtorDecl=FIR_MultiKernel_cincout(cint16 const ( & taps ) [ 4 ])  ClassCtorParams={ 'taps', 'cint16 const ( &) [ 4 ]', 'phi_1' }  KernelHeaderFile=FirDoubleStream.h  KernelClassName=DoubleStream::FIR_MultiKernel_cincout  KernelFunction=filter  KernelSourceFile=FirDoubleStream.cpp  KernelSearchPaths={'$SRC/aie_kernels'}  PreProcOptions={}  blockJsonConstraints="{\"type\":\"constraint\",\"constraintType\":\"location_kernel\",\"sid\":\"802\",\"lhs\":{\"type\":\"location\",\"templParam\":\"kernel\",\"args\":{\"type\":\"kernel\",\"name\":\"DualStreamSSR/SSR8/filter20\",\"sid\":\"802\"}},\"rhs\":{\"type\":\"tile\",\"args\":[{\"type\":\"evaluable\",\"expr\":\"27\",\"value\":27},{\"type\":\"evaluable\",\"expr\":\"3\",\"value\":3}]},\"equality\":true}"
      KernelAllAttrs=|
      | s[12;12;9;9;19;14;21;23;24;21;12;24;26;26;26;27;28;9;21;23;23;23;24;25;14;19;19;29]@FunctionNameDeclFileNamePortNamesPortTypesPortSerializedTypesPortDirectionsPortWindowSizeEnablesPortWindowMarginEnablesPortSynchronicityEnablesPortSignalSizeEnablesFunctionDeclFunctionTemplateSpecKindFunctionTemplateParamNamesFunctionTemplateParamKindsFunctionTemplateParamTypesFunctionTemplateParamValuesFunctionTemplateParamEnablesClassDeclClassTemplateSpecKindClassTemplateParamNamesClassTemplateParamKindsClassTemplateParamTypesClassTemplateParamValuesClassTemplateParamEnablesClassCtorDeclsClassCtorParamNamesClassCtorParamTypesClassCtorParamSerializedTypes[1 1]@C[28 1]@t6@filtert42@../../../aie/aie_kernels/FirDoubleStream.hC[4 1]@t4@sin1t4@sin2t3@cint4@coutC[4 1]@t30@input_stream_cint16 * restrictt30@input_stream_cint16 * restrictt26@input_stream< cacc48_t > *t27@output_stream< cacc48_t > *C[4 1]@t37@{Q2{P{Tinput_stream{1{t{Scint16}}}}}}t37@{Q2{P{Tinput_stream{1{t{Scint16}}}}}}t35@{P{Tinput_stream{1{t{Scacc48_t}}}}}t36@{P{Toutput_stream{1{t{Scacc48_t}}}}}C[4 1]@t5@inputt5@inputt5@inputt6@outputC[4 1]@l0@l0@l0@l0@C[4 1]@l0@l0@l0@l0@C[4 1]@l0@l0@l0@l0@C[4 1]@l0@l0@l0@l1@t281@namespace DoubleStream {
      | template < int NSamples, int ShiftAcc, bool DiscardSample, bool SwapRead > 
      | void FIR_MultiKernel_cincout::
      | filter(input_stream_cint16 * restrict sin1, input_stream_cint16 * restrict sin2, input_stream< cacc48_t > * cin, output_stream< cacc48_t > * cout);
      | }t4@nonee[0 1]@e[0 1]@e[0 1]@e[0 1]@e[0 1]@t132@namespace DoubleStream {
      | template < int NSamples, int ShiftAcc, bool DiscardSample, bool SwapRead > class FIR_MultiKernel_cincout;
      | }t8@implicitC[4 1]@t8@NSamplest8@ShiftAcct13@DiscardSamplet8@SwapReadC[4 1]@t7@nontypet7@nontypet7@nontypet7@nontypeC[4 1]@t3@intt3@intt4@boolt4@boolC[4 1]@nnnnC[4 1]@l1@l1@l1@l1@C[1 1]@t54@FIR_MultiKernel_cincout(cint16 const ( & taps ) [ 4 ])C[1 1]@C[1 1]@t4@tapsC[1 1]@C[1 1]@t23@cint16 const ( &) [ 4 ]C[1 1]@C[1 1]@t20@{R{Q1{C{Scint16}4}}}
      FunctionDecl=|
      | namespace DoubleStream {
      | template < int NSamples, int ShiftAcc, bool DiscardSample, bool SwapRead > 
      | void FIR_MultiKernel_cincout::
      | filter(input_stream_cint16 * restrict sin1, input_stream_cint16 * restrict sin2, input_stream< cacc48_t > * cin, output_stream< cacc48_t > * cout);
      | }
      ClassDeclTypeOptions=|
      | C[1 1]@t132@namespace DoubleStream {
      | template < int NSamples, int ShiftAcc, bool DiscardSample, bool SwapRead > class FIR_MultiKernel_cincout;
      | }
      ClassDecl=|
      | namespace DoubleStream {
      | template < int NSamples, int ShiftAcc, bool DiscardSample, bool SwapRead > class FIR_MultiKernel_cincout;
      | }
  filter21 : aieBasic/AIE Class Kernel  KernelAllAttrs=|  PortNames={'sin1'; 'sin2'; 'cin'; 'cout'}  PortSerializedTypes={'{Q2{P{Tinput_stream{1{t{Scint16}}}}}}'; '{Q2{P{Tinput_stream{1{t{Scint16}}}}}}'; '{P{Tinput_stream{1{t{Scacc48_t}}}}}'; '{P{Toutput_stream{1{t{Scacc48_t}}}}}'}  PortWindowSizes={0.000000000000000000e+00; 0.000000000000000000e+00; 0.000000000000000000e+00; 0.000000000000000000e+00}  PortWindowMargins={0.000000000000000000e+00; 0.000000000000000000e+00; 0.000000000000000000e+00; 0.000000000000000000e+00}  PortSynchronicities={'auto', 'auto', 'auto', 'auto'}  PortSignalSizes={0.000000000000000000e+00; 0.000000000000000000e+00; 0.000000000000000000e+00; 8.000000000000000000e+00}  ClassTemplateSpecKind=implicit  ClassTemplateParamNames={'NSamples'; 'ShiftAcc'; 'DiscardSample'; 'SwapRead'}  ClassTemplateParamKinds={'nontype'; 'nontype'; 'nontype'; 'nontype'}  ClassTemplateParamTypes={'int'; 'int'; 'bool'; 'bool'}  ClassTemplateParamValues={'512', '15', '0', '0'}  ClassCtorParamNames={'taps'}  ClassCtorParamSerializedTypes={'{R{Q1{C{Scint16}4}}}'}  ClassCtorParamValues={'[-21+26i 1183+239i 248-2878i -160+111i]'}  ClassIndex=1  ClassCtorIndex=1  ClassTabVisible=on  ClassTemplateParamsVisible=on  ClassCtorDeclVisible=on  ClassCtorParamsVisible=on  FunctionTabVisible=on  FunctionDecl=|  PortAttrs={ 'input', 'sin1', 'input_stream_cint16 * restrict', '', '', '', ''; 'input', 'sin2', 'input_stream_cint16 * restrict', '', '', '', ''; 'input', 'cin', 'input_stream< cacc48_t > *', '', '', '', ''; 'output', 'cout', 'output_stream< cacc48_t > *', '', '', '', 'OUTPUT_SIZE' }  PortAttrsEnables={'off', 'off', 'off', 'off', 'off', 'off', 'off';'off', 'off', 'off', 'off', 'off', 'off', 'off';'off', 'off', 'off', 'off', 'off', 'off', 'off';'off', 'off', 'off', 'off', 'off', 'off', 'on'}  SampleTime=-1  ClassDeclTypeOptions=|  ClassDecl=|  ClassTemplateParams={ 'NSamples', 'int', 'BURST_LENGTH'; 'ShiftAcc', 'int', 'SHIFT_ACC'; 'DiscardSample', 'bool', 'FALSE'; 'SwapRead', 'bool', 'FALSE' }  ClassTemplateParamsEnables={'off', 'off', 'on';'off', 'off', 'on';'off', 'off', 'on';'off', 'off', 'on'}  ClassCtorDeclTypeOptions=C[1 1]@t54@FIR_MultiKernel_cincout(cint16 const ( & taps ) [ 4 ])  ClassCtorDecl=FIR_MultiKernel_cincout(cint16 const ( & taps ) [ 4 ])  ClassCtorParams={ 'taps', 'cint16 const ( &) [ 4 ]', 'phi_2' }  KernelHeaderFile=FirDoubleStream.h  KernelClassName=DoubleStream::FIR_MultiKernel_cincout  KernelFunction=filter  KernelSourceFile=FirDoubleStream.cpp  KernelSearchPaths={'$SRC/aie_kernels'}  PreProcOptions={}  blockJsonConstraints="{\"type\":\"constraint\",\"constraintType\":\"location_kernel\",\"sid\":\"803\",\"lhs\":{\"type\":\"location\",\"templParam\":\"kernel\",\"args\":{\"type\":\"kernel\",\"name\":\"DualStreamSSR/SSR8/filter21\",\"sid\":\"803\"}},\"rhs\":{\"type\":\"tile\",\"args\":[{\"type\":\"evaluable\",\"expr\":\"28\",\"value\":28},{\"type\":\"evaluable\",\"expr\":\"3\",\"value\":3}]},\"equality\":true}"
      KernelAllAttrs=|
      | s[12;12;9;9;19;14;21;23;24;21;12;24;26;26;26;27;28;9;21;23;23;23;24;25;14;19;19;29]@FunctionNameDeclFileNamePortNamesPortTypesPortSerializedTypesPortDirectionsPortWindowSizeEnablesPortWindowMarginEnablesPortSynchronicityEnablesPortSignalSizeEnablesFunctionDeclFunctionTemplateSpecKindFunctionTemplateParamNamesFunctionTemplateParamKindsFunctionTemplateParamTypesFunctionTemplateParamValuesFunctionTemplateParamEnablesClassDeclClassTemplateSpecKindClassTemplateParamNamesClassTemplateParamKindsClassTemplateParamTypesClassTemplateParamValuesClassTemplateParamEnablesClassCtorDeclsClassCtorParamNamesClassCtorParamTypesClassCtorParamSerializedTypes[1 1]@C[28 1]@t6@filtert42@../../../aie/aie_kernels/FirDoubleStream.hC[4 1]@t4@sin1t4@sin2t3@cint4@coutC[4 1]@t30@input_stream_cint16 * restrictt30@input_stream_cint16 * restrictt26@input_stream< cacc48_t > *t27@output_stream< cacc48_t > *C[4 1]@t37@{Q2{P{Tinput_stream{1{t{Scint16}}}}}}t37@{Q2{P{Tinput_stream{1{t{Scint16}}}}}}t35@{P{Tinput_stream{1{t{Scacc48_t}}}}}t36@{P{Toutput_stream{1{t{Scacc48_t}}}}}C[4 1]@t5@inputt5@inputt5@inputt6@outputC[4 1]@l0@l0@l0@l0@C[4 1]@l0@l0@l0@l0@C[4 1]@l0@l0@l0@l0@C[4 1]@l0@l0@l0@l1@t281@namespace DoubleStream {
      | template < int NSamples, int ShiftAcc, bool DiscardSample, bool SwapRead > 
      | void FIR_MultiKernel_cincout::
      | filter(input_stream_cint16 * restrict sin1, input_stream_cint16 * restrict sin2, input_stream< cacc48_t > * cin, output_stream< cacc48_t > * cout);
      | }t4@nonee[0 1]@e[0 1]@e[0 1]@e[0 1]@e[0 1]@t132@namespace DoubleStream {
      | template < int NSamples, int ShiftAcc, bool DiscardSample, bool SwapRead > class FIR_MultiKernel_cincout;
      | }t8@implicitC[4 1]@t8@NSamplest8@ShiftAcct13@DiscardSamplet8@SwapReadC[4 1]@t7@nontypet7@nontypet7@nontypet7@nontypeC[4 1]@t3@intt3@intt4@boolt4@boolC[4 1]@nnnnC[4 1]@l1@l1@l1@l1@C[1 1]@t54@FIR_MultiKernel_cincout(cint16 const ( & taps ) [ 4 ])C[1 1]@C[1 1]@t4@tapsC[1 1]@C[1 1]@t23@cint16 const ( &) [ 4 ]C[1 1]@C[1 1]@t20@{R{Q1{C{Scint16}4}}}
      FunctionDecl=|
      | namespace DoubleStream {
      | template < int NSamples, int ShiftAcc, bool DiscardSample, bool SwapRead > 
      | void FIR_MultiKernel_cincout::
      | filter(input_stream_cint16 * restrict sin1, input_stream_cint16 * restrict sin2, input_stream< cacc48_t > * cin, output_stream< cacc48_t > * cout);
      | }
      ClassDeclTypeOptions=|
      | C[1 1]@t132@namespace DoubleStream {
      | template < int NSamples, int ShiftAcc, bool DiscardSample, bool SwapRead > class FIR_MultiKernel_cincout;
      | }
      ClassDecl=|
      | namespace DoubleStream {
      | template < int NSamples, int ShiftAcc, bool DiscardSample, bool SwapRead > class FIR_MultiKernel_cincout;
      | }
  filter22 : aieBasic/AIE Class Kernel  KernelAllAttrs=|  PortNames={'sin1'; 'sin2'; 'cin'; 'cout'}  PortSerializedTypes={'{Q2{P{Tinput_stream{1{t{Scint16}}}}}}'; '{Q2{P{Tinput_stream{1{t{Scint16}}}}}}'; '{P{Tinput_stream{1{t{Scacc48_t}}}}}'; '{P{Toutput_stream{1{t{Scacc48_t}}}}}'}  PortWindowSizes={0.000000000000000000e+00; 0.000000000000000000e+00; 0.000000000000000000e+00; 0.000000000000000000e+00}  PortWindowMargins={0.000000000000000000e+00; 0.000000000000000000e+00; 0.000000000000000000e+00; 0.000000000000000000e+00}  PortSynchronicities={'auto', 'auto', 'auto', 'auto'}  PortSignalSizes={0.000000000000000000e+00; 0.000000000000000000e+00; 0.000000000000000000e+00; 8.000000000000000000e+00}  ClassTemplateSpecKind=implicit  ClassTemplateParamNames={'NSamples'; 'ShiftAcc'; 'DiscardSample'; 'SwapRead'}  ClassTemplateParamKinds={'nontype'; 'nontype'; 'nontype'; 'nontype'}  ClassTemplateParamTypes={'int'; 'int'; 'bool'; 'bool'}  ClassTemplateParamValues={'512', '15', '1', '0'}  ClassCtorParamNames={'taps'}  ClassCtorParamSerializedTypes={'{R{Q1{C{Scint16}4}}}'}  ClassCtorParamValues={'[146-91i 4086+5221i 237-54i -83-21i]'}  ClassIndex=1  ClassCtorIndex=1  ClassTabVisible=on  ClassTemplateParamsVisible=on  ClassCtorDeclVisible=on  ClassCtorParamsVisible=on  FunctionTabVisible=on  FunctionDecl=|  PortAttrs={ 'input', 'sin1', 'input_stream_cint16 * restrict', '', '', '', ''; 'input', 'sin2', 'input_stream_cint16 * restrict', '', '', '', ''; 'input', 'cin', 'input_stream< cacc48_t > *', '', '', '', ''; 'output', 'cout', 'output_stream< cacc48_t > *', '', '', '', 'OUTPUT_SIZE' }  PortAttrsEnables={'off', 'off', 'off', 'off', 'off', 'off', 'off';'off', 'off', 'off', 'off', 'off', 'off', 'off';'off', 'off', 'off', 'off', 'off', 'off', 'off';'off', 'off', 'off', 'off', 'off', 'off', 'on'}  SampleTime=-1  ClassDeclTypeOptions=|  ClassDecl=|  ClassTemplateParams={ 'NSamples', 'int', 'BURST_LENGTH'; 'ShiftAcc', 'int', 'SHIFT_ACC'; 'DiscardSample', 'bool', 'TRUE'; 'SwapRead', 'bool', 'FALSE' }  ClassTemplateParamsEnables={'off', 'off', 'on';'off', 'off', 'on';'off', 'off', 'on';'off', 'off', 'on'}  ClassCtorDeclTypeOptions=C[1 1]@t54@FIR_MultiKernel_cincout(cint16 const ( & taps ) [ 4 ])  ClassCtorDecl=FIR_MultiKernel_cincout(cint16 const ( & taps ) [ 4 ])  ClassCtorParams={ 'taps', 'cint16 const ( &) [ 4 ]', 'phi_6' }  KernelHeaderFile=FirDoubleStream.h  KernelClassName=DoubleStream::FIR_MultiKernel_cincout  KernelFunction=filter  KernelSourceFile=FirDoubleStream.cpp  KernelSearchPaths={'$SRC/aie_kernels'}  PreProcOptions={}  blockJsonConstraints="{\"type\":\"constraint\",\"constraintType\":\"location_kernel\",\"sid\":\"804\",\"lhs\":{\"type\":\"location\",\"templParam\":\"kernel\",\"args\":{\"type\":\"kernel\",\"name\":\"DualStreamSSR/SSR8/filter22\",\"sid\":\"804\"}},\"rhs\":{\"type\":\"tile\",\"args\":[{\"type\":\"evaluable\",\"expr\":\"24\",\"value\":24},{\"type\":\"evaluable\",\"expr\":\"3\",\"value\":3}]},\"equality\":true}"
      KernelAllAttrs=|
      | s[12;12;9;9;19;14;21;23;24;21;12;24;26;26;26;27;28;9;21;23;23;23;24;25;14;19;19;29]@FunctionNameDeclFileNamePortNamesPortTypesPortSerializedTypesPortDirectionsPortWindowSizeEnablesPortWindowMarginEnablesPortSynchronicityEnablesPortSignalSizeEnablesFunctionDeclFunctionTemplateSpecKindFunctionTemplateParamNamesFunctionTemplateParamKindsFunctionTemplateParamTypesFunctionTemplateParamValuesFunctionTemplateParamEnablesClassDeclClassTemplateSpecKindClassTemplateParamNamesClassTemplateParamKindsClassTemplateParamTypesClassTemplateParamValuesClassTemplateParamEnablesClassCtorDeclsClassCtorParamNamesClassCtorParamTypesClassCtorParamSerializedTypes[1 1]@C[28 1]@t6@filtert42@../../../aie/aie_kernels/FirDoubleStream.hC[4 1]@t4@sin1t4@sin2t3@cint4@coutC[4 1]@t30@input_stream_cint16 * restrictt30@input_stream_cint16 * restrictt26@input_stream< cacc48_t > *t27@output_stream< cacc48_t > *C[4 1]@t37@{Q2{P{Tinput_stream{1{t{Scint16}}}}}}t37@{Q2{P{Tinput_stream{1{t{Scint16}}}}}}t35@{P{Tinput_stream{1{t{Scacc48_t}}}}}t36@{P{Toutput_stream{1{t{Scacc48_t}}}}}C[4 1]@t5@inputt5@inputt5@inputt6@outputC[4 1]@l0@l0@l0@l0@C[4 1]@l0@l0@l0@l0@C[4 1]@l0@l0@l0@l0@C[4 1]@l0@l0@l0@l1@t281@namespace DoubleStream {
      | template < int NSamples, int ShiftAcc, bool DiscardSample, bool SwapRead > 
      | void FIR_MultiKernel_cincout::
      | filter(input_stream_cint16 * restrict sin1, input_stream_cint16 * restrict sin2, input_stream< cacc48_t > * cin, output_stream< cacc48_t > * cout);
      | }t4@nonee[0 1]@e[0 1]@e[0 1]@e[0 1]@e[0 1]@t132@namespace DoubleStream {
      | template < int NSamples, int ShiftAcc, bool DiscardSample, bool SwapRead > class FIR_MultiKernel_cincout;
      | }t8@implicitC[4 1]@t8@NSamplest8@ShiftAcct13@DiscardSamplet8@SwapReadC[4 1]@t7@nontypet7@nontypet7@nontypet7@nontypeC[4 1]@t3@intt3@intt4@boolt4@boolC[4 1]@nnnnC[4 1]@l1@l1@l1@l1@C[1 1]@t54@FIR_MultiKernel_cincout(cint16 const ( & taps ) [ 4 ])C[1 1]@C[1 1]@t4@tapsC[1 1]@C[1 1]@t23@cint16 const ( &) [ 4 ]C[1 1]@C[1 1]@t20@{R{Q1{C{Scint16}4}}}
      FunctionDecl=|
      | namespace DoubleStream {
      | template < int NSamples, int ShiftAcc, bool DiscardSample, bool SwapRead > 
      | void FIR_MultiKernel_cincout::
      | filter(input_stream_cint16 * restrict sin1, input_stream_cint16 * restrict sin2, input_stream< cacc48_t > * cin, output_stream< cacc48_t > * cout);
      | }
      ClassDeclTypeOptions=|
      | C[1 1]@t132@namespace DoubleStream {
      | template < int NSamples, int ShiftAcc, bool DiscardSample, bool SwapRead > class FIR_MultiKernel_cincout;
      | }
      ClassDecl=|
      | namespace DoubleStream {
      | template < int NSamples, int ShiftAcc, bool DiscardSample, bool SwapRead > class FIR_MultiKernel_cincout;
      | }
  filter23 : aieBasic/AIE Class Kernel  KernelAllAttrs=|  PortNames={'sin1'; 'sin2'; 'cin'; 'sout1'; 'sout2'}  PortSerializedTypes={'{Q2{P{Tinput_stream{1{t{Scint16}}}}}}'; '{Q2{P{Tinput_stream{1{t{Scint16}}}}}}'; '{P{Tinput_stream{1{t{Scacc48_t}}}}}'; '{Q2{P{Toutput_stream{1{t{Scint16}}}}}}'; '{Q2{P{Toutput_stream{1{t{Scint16}}}}}}'}  PortWindowSizes={0.000000000000000000e+00; 0.000000000000000000e+00; 0.000000000000000000e+00; 0.000000000000000000e+00; 0.000000000000000000e+00}  PortWindowMargins={0.000000000000000000e+00; 0.000000000000000000e+00; 0.000000000000000000e+00; 0.000000000000000000e+00; 0.000000000000000000e+00}  PortSynchronicities={'auto', 'auto', 'auto', 'auto', 'auto'}  PortSignalSizes={0.000000000000000000e+00; 0.000000000000000000e+00; 0.000000000000000000e+00; 4.000000000000000000e+00; 4.000000000000000000e+00}  ClassTemplateSpecKind=implicit  ClassTemplateParamNames={'NSamples'; 'ShiftAcc'; 'DiscardSample'; 'SwapRead'}  ClassTemplateParamKinds={'nontype'; 'nontype'; 'nontype'; 'nontype'}  ClassTemplateParamTypes={'int'; 'int'; 'bool'; 'bool'}  ClassTemplateParamValues={'512', '15', '1', '0'}  ClassCtorParamNames={'taps'}  ClassCtorParamSerializedTypes={'{R{Q1{C{Scint16}4}}}'}  ClassCtorParamValues={'[-160-111i 248+2878i 1183-239i -21-26i]'}  ClassIndex=1  ClassCtorIndex=1  ClassTabVisible=on  ClassTemplateParamsVisible=on  ClassCtorDeclVisible=on  ClassCtorParamsVisible=on  FunctionTabVisible=on  FunctionDecl=|  PortAttrs={ 'input', 'sin1', 'input_stream_cint16 * restrict', '', '', '', ''; 'input', 'sin2', 'input_stream_cint16 * restrict', '', '', '', ''; 'input', 'cin', 'input_stream< cacc48_t > *', '', '', '', ''; 'output', 'sout1', 'output_stream_cint16 * restrict', '', '', '', 'OUTPUT_SIZE/2'; 'output', 'sout2', 'output_stream_cint16 * restrict', '', '', '', 'OUTPUT_SIZE/2' }  PortAttrsEnables={'off', 'off', 'off', 'off', 'off', 'off', 'off';'off', 'off', 'off', 'off', 'off', 'off', 'off';'off', 'off', 'off', 'off', 'off', 'off', 'off';'off', 'off', 'off', 'off', 'off', 'off', 'on';'off', 'off', 'off', 'off', 'off', 'off', 'on'}  SampleTime=-1  ClassDeclTypeOptions=|  ClassDecl=|  ClassTemplateParams={ 'NSamples', 'int', 'BURST_LENGTH'; 'ShiftAcc', 'int', 'SHIFT_ACC'; 'DiscardSample', 'bool', 'TRUE'; 'SwapRead', 'bool', 'FALSE' }  ClassTemplateParamsEnables={'off', 'off', 'on';'off', 'off', 'on';'off', 'off', 'on';'off', 'off', 'on'}  ClassCtorDeclTypeOptions=C[1 1]@t50@FIR_MultiKernel_cin(cint16 const ( & taps ) [ 4 ])  ClassCtorDecl=FIR_MultiKernel_cin(cint16 const ( & taps ) [ 4 ])  ClassCtorParams={ 'taps', 'cint16 const ( &) [ 4 ]', 'phi_5' }  KernelHeaderFile=FirDoubleStream.h  KernelClassName=DoubleStream::FIR_MultiKernel_cin  KernelFunction=filter  KernelSourceFile=FirDoubleStream.cpp  KernelSearchPaths={'$SRC/aie_kernels'}  PreProcOptions={}  blockJsonConstraints="{\"type\":\"constraint\",\"constraintType\":\"location_kernel\",\"sid\":\"805\",\"lhs\":{\"type\":\"location\",\"templParam\":\"kernel\",\"args\":{\"type\":\"kernel\",\"name\":\"DualStreamSSR/SSR8/filter23\",\"sid\":\"805\"}},\"rhs\":{\"type\":\"tile\",\"args\":[{\"type\":\"evaluable\",\"expr\":\"23\",\"value\":23},{\"type\":\"evaluable\",\"expr\":\"3\",\"value\":3}]},\"equality\":true}"
      KernelAllAttrs=|
      | s[12;12;9;9;19;14;21;23;24;21;12;24;26;26;26;27;28;9;21;23;23;23;24;25;14;19;19;29]@FunctionNameDeclFileNamePortNamesPortTypesPortSerializedTypesPortDirectionsPortWindowSizeEnablesPortWindowMarginEnablesPortSynchronicityEnablesPortSignalSizeEnablesFunctionDeclFunctionTemplateSpecKindFunctionTemplateParamNamesFunctionTemplateParamKindsFunctionTemplateParamTypesFunctionTemplateParamValuesFunctionTemplateParamEnablesClassDeclClassTemplateSpecKindClassTemplateParamNamesClassTemplateParamKindsClassTemplateParamTypesClassTemplateParamValuesClassTemplateParamEnablesClassCtorDeclsClassCtorParamNamesClassCtorParamTypesClassCtorParamSerializedTypes[1 1]@C[28 1]@t6@filtert42@../../../aie/aie_kernels/FirDoubleStream.hC[5 1]@t4@sin1t4@sin2t3@cint5@sout1t5@sout2C[5 1]@t30@input_stream_cint16 * restrictt30@input_stream_cint16 * restrictt26@input_stream< cacc48_t > *t31@output_stream_cint16 * restrictt31@output_stream_cint16 * restrictC[5 1]@t37@{Q2{P{Tinput_stream{1{t{Scint16}}}}}}t37@{Q2{P{Tinput_stream{1{t{Scint16}}}}}}t35@{P{Tinput_stream{1{t{Scacc48_t}}}}}t38@{Q2{P{Toutput_stream{1{t{Scint16}}}}}}t38@{Q2{P{Toutput_stream{1{t{Scint16}}}}}}C[5 1]@t5@inputt5@inputt5@inputt6@outputt6@outputC[5 1]@l0@l0@l0@l0@l0@C[5 1]@l0@l0@l0@l0@l0@C[5 1]@l0@l0@l0@l0@l0@C[5 1]@l0@l0@l0@l1@l1@t321@namespace DoubleStream {
      | template < int NSamples, int ShiftAcc, bool DiscardSample, bool SwapRead > 
      | void FIR_MultiKernel_cin::
      | filter(input_stream_cint16 * restrict sin1, input_stream_cint16 * restrict sin2, input_stream< cacc48_t > * cin, output_stream_cint16 * restrict sout1, output_stream_cint16 * restrict sout2);
      | }t4@nonee[0 1]@e[0 1]@e[0 1]@e[0 1]@e[0 1]@t128@namespace DoubleStream {
      | template < int NSamples, int ShiftAcc, bool DiscardSample, bool SwapRead > class FIR_MultiKernel_cin;
      | }t8@implicitC[4 1]@t8@NSamplest8@ShiftAcct13@DiscardSamplet8@SwapReadC[4 1]@t7@nontypet7@nontypet7@nontypet7@nontypeC[4 1]@t3@intt3@intt4@boolt4@boolC[4 1]@nnnnC[4 1]@l1@l1@l1@l1@C[1 1]@t50@FIR_MultiKernel_cin(cint16 const ( & taps ) [ 4 ])C[1 1]@C[1 1]@t4@tapsC[1 1]@C[1 1]@t23@cint16 const ( &) [ 4 ]C[1 1]@C[1 1]@t20@{R{Q1{C{Scint16}4}}}
      FunctionDecl=|
      | namespace DoubleStream {
      | template < int NSamples, int ShiftAcc, bool DiscardSample, bool SwapRead > 
      | void FIR_MultiKernel_cin::
      | filter(input_stream_cint16 * restrict sin1, input_stream_cint16 * restrict sin2, input_stream< cacc48_t > * cin, output_stream_cint16 * restrict sout1, output_stream_cint16 * restrict sout2);
      | }
      ClassDeclTypeOptions=|
      | C[1 1]@t128@namespace DoubleStream {
      | template < int NSamples, int ShiftAcc, bool DiscardSample, bool SwapRead > class FIR_MultiKernel_cin;
      | }
      ClassDecl=|
      | namespace DoubleStream {
      | template < int NSamples, int ShiftAcc, bool DiscardSample, bool SwapRead > class FIR_MultiKernel_cin;
      | }
  filter24 : aieBasic/AIE Class Kernel  KernelAllAttrs=|  PortNames={'sin1'; 'sin2'; 'cin'; 'cout'}  PortSerializedTypes={'{Q2{P{Tinput_stream{1{t{Scint16}}}}}}'; '{Q2{P{Tinput_stream{1{t{Scint16}}}}}}'; '{P{Tinput_stream{1{t{Scacc48_t}}}}}'; '{P{Toutput_stream{1{t{Scacc48_t}}}}}'}  PortWindowSizes={0.000000000000000000e+00; 0.000000000000000000e+00; 0.000000000000000000e+00; 0.000000000000000000e+00}  PortWindowMargins={0.000000000000000000e+00; 0.000000000000000000e+00; 0.000000000000000000e+00; 0.000000000000000000e+00}  PortSynchronicities={'auto', 'auto', 'auto', 'auto'}  PortSignalSizes={0.000000000000000000e+00; 0.000000000000000000e+00; 0.000000000000000000e+00; 8.000000000000000000e+00}  ClassTemplateSpecKind=implicit  ClassTemplateParamNames={'NSamples'; 'ShiftAcc'; 'DiscardSample'; 'SwapRead'}  ClassTemplateParamKinds={'nontype'; 'nontype'; 'nontype'; 'nontype'}  ClassTemplateParamTypes={'int'; 'int'; 'bool'; 'bool'}  ClassTemplateParamValues={'512', '15', '0', '0'}  ClassCtorParamNames={'taps'}  ClassCtorParamSerializedTypes={'{R{Q1{C{Scint16}4}}}'}  ClassCtorParamValues={'[-54-21i 102-525i 8773-2748i 342+439i]'}  ClassIndex=1  ClassCtorIndex=1  ClassTabVisible=on  ClassTemplateParamsVisible=on  ClassCtorDeclVisible=on  ClassCtorParamsVisible=on  FunctionTabVisible=on  FunctionDecl=|  PortAttrs={ 'input', 'sin1', 'input_stream_cint16 * restrict', '', '', '', ''; 'input', 'sin2', 'input_stream_cint16 * restrict', '', '', '', ''; 'input', 'cin', 'input_stream< cacc48_t > *', '', '', '', ''; 'output', 'cout', 'output_stream< cacc48_t > *', '', '', '', 'OUTPUT_SIZE' }  PortAttrsEnables={'off', 'off', 'off', 'off', 'off', 'off', 'off';'off', 'off', 'off', 'off', 'off', 'off', 'off';'off', 'off', 'off', 'off', 'off', 'off', 'off';'off', 'off', 'off', 'off', 'off', 'off', 'on'}  SampleTime=-1  ClassDeclTypeOptions=|  ClassDecl=|  ClassTemplateParams={ 'NSamples', 'int', 'BURST_LENGTH'; 'ShiftAcc', 'int', 'SHIFT_ACC'; 'DiscardSample', 'bool', 'FALSE'; 'SwapRead', 'bool', 'FALSE' }  ClassTemplateParamsEnables={'off', 'off', 'on';'off', 'off', 'on';'off', 'off', 'on';'off', 'off', 'on'}  ClassCtorDeclTypeOptions=C[1 1]@t54@FIR_MultiKernel_cincout(cint16 const ( & taps ) [ 4 ])  ClassCtorDecl=FIR_MultiKernel_cincout(cint16 const ( & taps ) [ 4 ])  ClassCtorParams={ 'taps', 'cint16 const ( &) [ 4 ]', 'phi_0' }  KernelHeaderFile=FirDoubleStream.h  KernelClassName=DoubleStream::FIR_MultiKernel_cincout  KernelFunction=filter  KernelSourceFile=FirDoubleStream.cpp  KernelSearchPaths={'$SRC/aie_kernels'}  PreProcOptions={}  blockJsonConstraints="{\"type\":\"constraint\",\"constraintType\":\"location_kernel\",\"sid\":\"806\",\"lhs\":{\"type\":\"location\",\"templParam\":\"kernel\",\"args\":{\"type\":\"kernel\",\"name\":\"DualStreamSSR/SSR8/filter24\",\"sid\":\"806\"}},\"rhs\":{\"type\":\"tile\",\"args\":[{\"type\":\"evaluable\",\"expr\":\"25\",\"value\":25},{\"type\":\"evaluable\",\"expr\":\"2\",\"value\":2}]},\"equality\":true}"
      KernelAllAttrs=|
      | s[12;12;9;9;19;14;21;23;24;21;12;24;26;26;26;27;28;9;21;23;23;23;24;25;14;19;19;29]@FunctionNameDeclFileNamePortNamesPortTypesPortSerializedTypesPortDirectionsPortWindowSizeEnablesPortWindowMarginEnablesPortSynchronicityEnablesPortSignalSizeEnablesFunctionDeclFunctionTemplateSpecKindFunctionTemplateParamNamesFunctionTemplateParamKindsFunctionTemplateParamTypesFunctionTemplateParamValuesFunctionTemplateParamEnablesClassDeclClassTemplateSpecKindClassTemplateParamNamesClassTemplateParamKindsClassTemplateParamTypesClassTemplateParamValuesClassTemplateParamEnablesClassCtorDeclsClassCtorParamNamesClassCtorParamTypesClassCtorParamSerializedTypes[1 1]@C[28 1]@t6@filtert42@../../../aie/aie_kernels/FirDoubleStream.hC[4 1]@t4@sin1t4@sin2t3@cint4@coutC[4 1]@t30@input_stream_cint16 * restrictt30@input_stream_cint16 * restrictt26@input_stream< cacc48_t > *t27@output_stream< cacc48_t > *C[4 1]@t37@{Q2{P{Tinput_stream{1{t{Scint16}}}}}}t37@{Q2{P{Tinput_stream{1{t{Scint16}}}}}}t35@{P{Tinput_stream{1{t{Scacc48_t}}}}}t36@{P{Toutput_stream{1{t{Scacc48_t}}}}}C[4 1]@t5@inputt5@inputt5@inputt6@outputC[4 1]@l0@l0@l0@l0@C[4 1]@l0@l0@l0@l0@C[4 1]@l0@l0@l0@l0@C[4 1]@l0@l0@l0@l1@t281@namespace DoubleStream {
      | template < int NSamples, int ShiftAcc, bool DiscardSample, bool SwapRead > 
      | void FIR_MultiKernel_cincout::
      | filter(input_stream_cint16 * restrict sin1, input_stream_cint16 * restrict sin2, input_stream< cacc48_t > * cin, output_stream< cacc48_t > * cout);
      | }t4@nonee[0 1]@e[0 1]@e[0 1]@e[0 1]@e[0 1]@t132@namespace DoubleStream {
      | template < int NSamples, int ShiftAcc, bool DiscardSample, bool SwapRead > class FIR_MultiKernel_cincout;
      | }t8@implicitC[4 1]@t8@NSamplest8@ShiftAcct13@DiscardSamplet8@SwapReadC[4 1]@t7@nontypet7@nontypet7@nontypet7@nontypeC[4 1]@t3@intt3@intt4@boolt4@boolC[4 1]@nnnnC[4 1]@l1@l1@l1@l1@C[1 1]@t54@FIR_MultiKernel_cincout(cint16 const ( & taps ) [ 4 ])C[1 1]@C[1 1]@t4@tapsC[1 1]@C[1 1]@t23@cint16 const ( &) [ 4 ]C[1 1]@C[1 1]@t20@{R{Q1{C{Scint16}4}}}
      FunctionDecl=|
      | namespace DoubleStream {
      | template < int NSamples, int ShiftAcc, bool DiscardSample, bool SwapRead > 
      | void FIR_MultiKernel_cincout::
      | filter(input_stream_cint16 * restrict sin1, input_stream_cint16 * restrict sin2, input_stream< cacc48_t > * cin, output_stream< cacc48_t > * cout);
      | }
      ClassDeclTypeOptions=|
      | C[1 1]@t132@namespace DoubleStream {
      | template < int NSamples, int ShiftAcc, bool DiscardSample, bool SwapRead > class FIR_MultiKernel_cincout;
      | }
      ClassDecl=|
      | namespace DoubleStream {
      | template < int NSamples, int ShiftAcc, bool DiscardSample, bool SwapRead > class FIR_MultiKernel_cincout;
      | }
  filter25 : aieBasic/AIE Class Kernel  KernelAllAttrs=|  PortNames={'sin1'; 'sin2'; 'cin'; 'cout'}  PortSerializedTypes={'{Q2{P{Tinput_stream{1{t{Scint16}}}}}}'; '{Q2{P{Tinput_stream{1{t{Scint16}}}}}}'; '{P{Tinput_stream{1{t{Scacc48_t}}}}}'; '{P{Toutput_stream{1{t{Scacc48_t}}}}}'}  PortWindowSizes={0.000000000000000000e+00; 0.000000000000000000e+00; 0.000000000000000000e+00; 0.000000000000000000e+00}  PortWindowMargins={0.000000000000000000e+00; 0.000000000000000000e+00; 0.000000000000000000e+00; 0.000000000000000000e+00}  PortSynchronicities={'auto', 'auto', 'auto', 'auto'}  PortSignalSizes={0.000000000000000000e+00; 0.000000000000000000e+00; 0.000000000000000000e+00; 8.000000000000000000e+00}  ClassTemplateSpecKind=implicit  ClassTemplateParamNames={'NSamples'; 'ShiftAcc'; 'DiscardSample'; 'SwapRead'}  ClassTemplateParamKinds={'nontype'; 'nontype'; 'nontype'; 'nontype'}  ClassTemplateParamTypes={'int'; 'int'; 'bool'; 'bool'}  ClassTemplateParamValues={'512', '15', '0', '0'}  ClassCtorParamNames={'taps'}  ClassCtorParamSerializedTypes={'{R{Q1{C{Scint16}4}}}'}  ClassCtorParamValues={'[-83+21i 237+54i 4086-5221i 146+91i]'}  ClassIndex=1  ClassCtorIndex=1  ClassTabVisible=on  ClassTemplateParamsVisible=on  ClassCtorDeclVisible=on  ClassCtorParamsVisible=on  FunctionTabVisible=on  FunctionDecl=|  PortAttrs={ 'input', 'sin1', 'input_stream_cint16 * restrict', '', '', '', ''; 'input', 'sin2', 'input_stream_cint16 * restrict', '', '', '', ''; 'input', 'cin', 'input_stream< cacc48_t > *', '', '', '', ''; 'output', 'cout', 'output_stream< cacc48_t > *', '', '', '', 'OUTPUT_SIZE' }  PortAttrsEnables={'off', 'off', 'off', 'off', 'off', 'off', 'off';'off', 'off', 'off', 'off', 'off', 'off', 'off';'off', 'off', 'off', 'off', 'off', 'off', 'off';'off', 'off', 'off', 'off', 'off', 'off', 'on'}  SampleTime=-1  ClassDeclTypeOptions=|  ClassDecl=|  ClassTemplateParams={ 'NSamples', 'int', 'BURST_LENGTH'; 'ShiftAcc', 'int', 'SHIFT_ACC'; 'DiscardSample', 'bool', 'FALSE'; 'SwapRead', 'bool', 'FALSE' }  ClassTemplateParamsEnables={'off', 'off', 'on';'off', 'off', 'on';'off', 'off', 'on';'off', 'off', 'on'}  ClassCtorDeclTypeOptions=C[1 1]@t54@FIR_MultiKernel_cincout(cint16 const ( & taps ) [ 4 ])  ClassCtorDecl=FIR_MultiKernel_cincout(cint16 const ( & taps ) [ 4 ])  ClassCtorParams={ 'taps', 'cint16 const ( &) [ 4 ]', 'phi_1' }  KernelHeaderFile=FirDoubleStream.h  KernelClassName=DoubleStream::FIR_MultiKernel_cincout  KernelFunction=filter  KernelSourceFile=FirDoubleStream.cpp  KernelSearchPaths={'$SRC/aie_kernels'}  PreProcOptions={}  blockJsonConstraints="{\"type\":\"constraint\",\"constraintType\":\"location_kernel\",\"sid\":\"807\",\"lhs\":{\"type\":\"location\",\"templParam\":\"kernel\",\"args\":{\"type\":\"kernel\",\"name\":\"DualStreamSSR/SSR8/filter25\",\"sid\":\"807\"}},\"rhs\":{\"type\":\"tile\",\"args\":[{\"type\":\"evaluable\",\"expr\":\"26\",\"value\":26},{\"type\":\"evaluable\",\"expr\":\"2\",\"value\":2}]},\"equality\":true}"
      KernelAllAttrs=|
      | s[12;12;9;9;19;14;21;23;24;21;12;24;26;26;26;27;28;9;21;23;23;23;24;25;14;19;19;29]@FunctionNameDeclFileNamePortNamesPortTypesPortSerializedTypesPortDirectionsPortWindowSizeEnablesPortWindowMarginEnablesPortSynchronicityEnablesPortSignalSizeEnablesFunctionDeclFunctionTemplateSpecKindFunctionTemplateParamNamesFunctionTemplateParamKindsFunctionTemplateParamTypesFunctionTemplateParamValuesFunctionTemplateParamEnablesClassDeclClassTemplateSpecKindClassTemplateParamNamesClassTemplateParamKindsClassTemplateParamTypesClassTemplateParamValuesClassTemplateParamEnablesClassCtorDeclsClassCtorParamNamesClassCtorParamTypesClassCtorParamSerializedTypes[1 1]@C[28 1]@t6@filtert42@../../../aie/aie_kernels/FirDoubleStream.hC[4 1]@t4@sin1t4@sin2t3@cint4@coutC[4 1]@t30@input_stream_cint16 * restrictt30@input_stream_cint16 * restrictt26@input_stream< cacc48_t > *t27@output_stream< cacc48_t > *C[4 1]@t37@{Q2{P{Tinput_stream{1{t{Scint16}}}}}}t37@{Q2{P{Tinput_stream{1{t{Scint16}}}}}}t35@{P{Tinput_stream{1{t{Scacc48_t}}}}}t36@{P{Toutput_stream{1{t{Scacc48_t}}}}}C[4 1]@t5@inputt5@inputt5@inputt6@outputC[4 1]@l0@l0@l0@l0@C[4 1]@l0@l0@l0@l0@C[4 1]@l0@l0@l0@l0@C[4 1]@l0@l0@l0@l1@t281@namespace DoubleStream {
      | template < int NSamples, int ShiftAcc, bool DiscardSample, bool SwapRead > 
      | void FIR_MultiKernel_cincout::
      | filter(input_stream_cint16 * restrict sin1, input_stream_cint16 * restrict sin2, input_stream< cacc48_t > * cin, output_stream< cacc48_t > * cout);
      | }t4@nonee[0 1]@e[0 1]@e[0 1]@e[0 1]@e[0 1]@t132@namespace DoubleStream {
      | template < int NSamples, int ShiftAcc, bool DiscardSample, bool SwapRead > class FIR_MultiKernel_cincout;
      | }t8@implicitC[4 1]@t8@NSamplest8@ShiftAcct13@DiscardSamplet8@SwapReadC[4 1]@t7@nontypet7@nontypet7@nontypet7@nontypeC[4 1]@t3@intt3@intt4@boolt4@boolC[4 1]@nnnnC[4 1]@l1@l1@l1@l1@C[1 1]@t54@FIR_MultiKernel_cincout(cint16 const ( & taps ) [ 4 ])C[1 1]@C[1 1]@t4@tapsC[1 1]@C[1 1]@t23@cint16 const ( &) [ 4 ]C[1 1]@C[1 1]@t20@{R{Q1{C{Scint16}4}}}
      FunctionDecl=|
      | namespace DoubleStream {
      | template < int NSamples, int ShiftAcc, bool DiscardSample, bool SwapRead > 
      | void FIR_MultiKernel_cincout::
      | filter(input_stream_cint16 * restrict sin1, input_stream_cint16 * restrict sin2, input_stream< cacc48_t > * cin, output_stream< cacc48_t > * cout);
      | }
      ClassDeclTypeOptions=|
      | C[1 1]@t132@namespace DoubleStream {
      | template < int NSamples, int ShiftAcc, bool DiscardSample, bool SwapRead > class FIR_MultiKernel_cincout;
      | }
      ClassDecl=|
      | namespace DoubleStream {
      | template < int NSamples, int ShiftAcc, bool DiscardSample, bool SwapRead > class FIR_MultiKernel_cincout;
      | }
  filter26 : aieBasic/AIE Class Kernel  KernelAllAttrs=|  PortNames={'sin1'; 'sin2'; 'cin'; 'cout'}  PortSerializedTypes={'{Q2{P{Tinput_stream{1{t{Scint16}}}}}}'; '{Q2{P{Tinput_stream{1{t{Scint16}}}}}}'; '{P{Tinput_stream{1{t{Scacc48_t}}}}}'; '{P{Toutput_stream{1{t{Scacc48_t}}}}}'}  PortWindowSizes={0.000000000000000000e+00; 0.000000000000000000e+00; 0.000000000000000000e+00; 0.000000000000000000e+00}  PortWindowMargins={0.000000000000000000e+00; 0.000000000000000000e+00; 0.000000000000000000e+00; 0.000000000000000000e+00}  PortSynchronicities={'auto', 'auto', 'auto', 'auto'}  PortSignalSizes={0.000000000000000000e+00; 0.000000000000000000e+00; 0.000000000000000000e+00; 8.000000000000000000e+00}  ClassTemplateSpecKind=implicit  ClassTemplateParamNames={'NSamples'; 'ShiftAcc'; 'DiscardSample'; 'SwapRead'}  ClassTemplateParamKinds={'nontype'; 'nontype'; 'nontype'; 'nontype'}  ClassTemplateParamTypes={'int'; 'int'; 'bool'; 'bool'}  ClassTemplateParamValues={'512', '15', '0', '0'}  ClassCtorParamNames={'taps'}  ClassCtorParamSerializedTypes={'{R{Q1{C{Scint16}4}}}'}  ClassCtorParamValues={'[-21+26i 1183+239i 248-2878i -160+111i]'}  ClassIndex=1  ClassCtorIndex=1  ClassTabVisible=on  ClassTemplateParamsVisible=on  ClassCtorDeclVisible=on  ClassCtorParamsVisible=on  FunctionTabVisible=on  FunctionDecl=|  PortAttrs={ 'input', 'sin1', 'input_stream_cint16 * restrict', '', '', '', ''; 'input', 'sin2', 'input_stream_cint16 * restrict', '', '', '', ''; 'input', 'cin', 'input_stream< cacc48_t > *', '', '', '', ''; 'output', 'cout', 'output_stream< cacc48_t > *', '', '', '', 'OUTPUT_SIZE' }  PortAttrsEnables={'off', 'off', 'off', 'off', 'off', 'off', 'off';'off', 'off', 'off', 'off', 'off', 'off', 'off';'off', 'off', 'off', 'off', 'off', 'off', 'off';'off', 'off', 'off', 'off', 'off', 'off', 'on'}  SampleTime=-1  ClassDeclTypeOptions=|  ClassDecl=|  ClassTemplateParams={ 'NSamples', 'int', 'BURST_LENGTH'; 'ShiftAcc', 'int', 'SHIFT_ACC'; 'DiscardSample', 'bool', 'FALSE'; 'SwapRead', 'bool', 'FALSE' }  ClassTemplateParamsEnables={'off', 'off', 'on';'off', 'off', 'on';'off', 'off', 'on';'off', 'off', 'on'}  ClassCtorDeclTypeOptions=C[1 1]@t54@FIR_MultiKernel_cincout(cint16 const ( & taps ) [ 4 ])  ClassCtorDecl=FIR_MultiKernel_cincout(cint16 const ( & taps ) [ 4 ])  ClassCtorParams={ 'taps', 'cint16 const ( &) [ 4 ]', 'phi_2' }  KernelHeaderFile=FirDoubleStream.h  KernelClassName=DoubleStream::FIR_MultiKernel_cincout  KernelFunction=filter  KernelSourceFile=FirDoubleStream.cpp  KernelSearchPaths={'$SRC/aie_kernels'}  PreProcOptions={}  blockJsonConstraints="{\"type\":\"constraint\",\"constraintType\":\"location_kernel\",\"sid\":\"808\",\"lhs\":{\"type\":\"location\",\"templParam\":\"kernel\",\"args\":{\"type\":\"kernel\",\"name\":\"DualStreamSSR/SSR8/filter26\",\"sid\":\"808\"}},\"rhs\":{\"type\":\"tile\",\"args\":[{\"type\":\"evaluable\",\"expr\":\"27\",\"value\":27},{\"type\":\"evaluable\",\"expr\":\"2\",\"value\":2}]},\"equality\":true}"
      KernelAllAttrs=|
      | s[12;12;9;9;19;14;21;23;24;21;12;24;26;26;26;27;28;9;21;23;23;23;24;25;14;19;19;29]@FunctionNameDeclFileNamePortNamesPortTypesPortSerializedTypesPortDirectionsPortWindowSizeEnablesPortWindowMarginEnablesPortSynchronicityEnablesPortSignalSizeEnablesFunctionDeclFunctionTemplateSpecKindFunctionTemplateParamNamesFunctionTemplateParamKindsFunctionTemplateParamTypesFunctionTemplateParamValuesFunctionTemplateParamEnablesClassDeclClassTemplateSpecKindClassTemplateParamNamesClassTemplateParamKindsClassTemplateParamTypesClassTemplateParamValuesClassTemplateParamEnablesClassCtorDeclsClassCtorParamNamesClassCtorParamTypesClassCtorParamSerializedTypes[1 1]@C[28 1]@t6@filtert42@../../../aie/aie_kernels/FirDoubleStream.hC[4 1]@t4@sin1t4@sin2t3@cint4@coutC[4 1]@t30@input_stream_cint16 * restrictt30@input_stream_cint16 * restrictt26@input_stream< cacc48_t > *t27@output_stream< cacc48_t > *C[4 1]@t37@{Q2{P{Tinput_stream{1{t{Scint16}}}}}}t37@{Q2{P{Tinput_stream{1{t{Scint16}}}}}}t35@{P{Tinput_stream{1{t{Scacc48_t}}}}}t36@{P{Toutput_stream{1{t{Scacc48_t}}}}}C[4 1]@t5@inputt5@inputt5@inputt6@outputC[4 1]@l0@l0@l0@l0@C[4 1]@l0@l0@l0@l0@C[4 1]@l0@l0@l0@l0@C[4 1]@l0@l0@l0@l1@t281@namespace DoubleStream {
      | template < int NSamples, int ShiftAcc, bool DiscardSample, bool SwapRead > 
      | void FIR_MultiKernel_cincout::
      | filter(input_stream_cint16 * restrict sin1, input_stream_cint16 * restrict sin2, input_stream< cacc48_t > * cin, output_stream< cacc48_t > * cout);
      | }t4@nonee[0 1]@e[0 1]@e[0 1]@e[0 1]@e[0 1]@t132@namespace DoubleStream {
      | template < int NSamples, int ShiftAcc, bool DiscardSample, bool SwapRead > class FIR_MultiKernel_cincout;
      | }t8@implicitC[4 1]@t8@NSamplest8@ShiftAcct13@DiscardSamplet8@SwapReadC[4 1]@t7@nontypet7@nontypet7@nontypet7@nontypeC[4 1]@t3@intt3@intt4@boolt4@boolC[4 1]@nnnnC[4 1]@l1@l1@l1@l1@C[1 1]@t54@FIR_MultiKernel_cincout(cint16 const ( & taps ) [ 4 ])C[1 1]@C[1 1]@t4@tapsC[1 1]@C[1 1]@t23@cint16 const ( &) [ 4 ]C[1 1]@C[1 1]@t20@{R{Q1{C{Scint16}4}}}
      FunctionDecl=|
      | namespace DoubleStream {
      | template < int NSamples, int ShiftAcc, bool DiscardSample, bool SwapRead > 
      | void FIR_MultiKernel_cincout::
      | filter(input_stream_cint16 * restrict sin1, input_stream_cint16 * restrict sin2, input_stream< cacc48_t > * cin, output_stream< cacc48_t > * cout);
      | }
      ClassDeclTypeOptions=|
      | C[1 1]@t132@namespace DoubleStream {
      | template < int NSamples, int ShiftAcc, bool DiscardSample, bool SwapRead > class FIR_MultiKernel_cincout;
      | }
      ClassDecl=|
      | namespace DoubleStream {
      | template < int NSamples, int ShiftAcc, bool DiscardSample, bool SwapRead > class FIR_MultiKernel_cincout;
      | }
  filter27 : aieBasic/AIE Class Kernel  KernelAllAttrs=|  PortNames={'sin1'; 'sin2'; 'cin'; 'cout'}  PortSerializedTypes={'{Q2{P{Tinput_stream{1{t{Scint16}}}}}}'; '{Q2{P{Tinput_stream{1{t{Scint16}}}}}}'; '{P{Tinput_stream{1{t{Scacc48_t}}}}}'; '{P{Toutput_stream{1{t{Scacc48_t}}}}}'}  PortWindowSizes={0.000000000000000000e+00; 0.000000000000000000e+00; 0.000000000000000000e+00; 0.000000000000000000e+00}  PortWindowMargins={0.000000000000000000e+00; 0.000000000000000000e+00; 0.000000000000000000e+00; 0.000000000000000000e+00}  PortSynchronicities={'auto', 'auto', 'auto', 'auto'}  PortSignalSizes={0.000000000000000000e+00; 0.000000000000000000e+00; 0.000000000000000000e+00; 8.000000000000000000e+00}  ClassTemplateSpecKind=implicit  ClassTemplateParamNames={'NSamples'; 'ShiftAcc'; 'DiscardSample'; 'SwapRead'}  ClassTemplateParamKinds={'nontype'; 'nontype'; 'nontype'; 'nontype'}  ClassTemplateParamTypes={'int'; 'int'; 'bool'; 'bool'}  ClassTemplateParamValues={'512', '15', '0', '0'}  ClassCtorParamNames={'taps'}  ClassCtorParamSerializedTypes={'{R{Q1{C{Scint16}4}}}'}  ClassCtorParamValues={'[14-121i 1454-497i 237+96i -121+233i]'}  ClassIndex=1  ClassCtorIndex=1  ClassTabVisible=on  ClassTemplateParamsVisible=on  ClassCtorDeclVisible=on  ClassCtorParamsVisible=on  FunctionTabVisible=on  FunctionDecl=|  PortAttrs={ 'input', 'sin1', 'input_stream_cint16 * restrict', '', '', '', ''; 'input', 'sin2', 'input_stream_cint16 * restrict', '', '', '', ''; 'input', 'cin', 'input_stream< cacc48_t > *', '', '', '', ''; 'output', 'cout', 'output_stream< cacc48_t > *', '', '', '', 'OUTPUT_SIZE' }  PortAttrsEnables={'off', 'off', 'off', 'off', 'off', 'off', 'off';'off', 'off', 'off', 'off', 'off', 'off', 'off';'off', 'off', 'off', 'off', 'off', 'off', 'off';'off', 'off', 'off', 'off', 'off', 'off', 'on'}  SampleTime=-1  ClassDeclTypeOptions=|  ClassDecl=|  ClassTemplateParams={ 'NSamples', 'int', 'BURST_LENGTH'; 'ShiftAcc', 'int', 'SHIFT_ACC'; 'DiscardSample', 'bool', 'FALSE'; 'SwapRead', 'bool', 'FALSE' }  ClassTemplateParamsEnables={'off', 'off', 'on';'off', 'off', 'on';'off', 'off', 'on';'off', 'off', 'on'}  ClassCtorDeclTypeOptions=C[1 1]@t54@FIR_MultiKernel_cincout(cint16 const ( & taps ) [ 4 ])  ClassCtorDecl=FIR_MultiKernel_cincout(cint16 const ( & taps ) [ 4 ])  ClassCtorParams={ 'taps', 'cint16 const ( &) [ 4 ]', 'phi_3' }  KernelHeaderFile=FirDoubleStream.h  KernelClassName=DoubleStream::FIR_MultiKernel_cincout  KernelFunction=filter  KernelSourceFile=FirDoubleStream.cpp  KernelSearchPaths={'$SRC/aie_kernels'}  PreProcOptions={}  blockJsonConstraints="{\"type\":\"constraint\",\"constraintType\":\"location_kernel\",\"sid\":\"809\",\"lhs\":{\"type\":\"location\",\"templParam\":\"kernel\",\"args\":{\"type\":\"kernel\",\"name\":\"DualStreamSSR/SSR8/filter27\",\"sid\":\"809\"}},\"rhs\":{\"type\":\"tile\",\"args\":[{\"type\":\"evaluable\",\"expr\":\"28\",\"value\":28},{\"type\":\"evaluable\",\"expr\":\"2\",\"value\":2}]},\"equality\":true}"
      KernelAllAttrs=|
      | s[12;12;9;9;19;14;21;23;24;21;12;24;26;26;26;27;28;9;21;23;23;23;24;25;14;19;19;29]@FunctionNameDeclFileNamePortNamesPortTypesPortSerializedTypesPortDirectionsPortWindowSizeEnablesPortWindowMarginEnablesPortSynchronicityEnablesPortSignalSizeEnablesFunctionDeclFunctionTemplateSpecKindFunctionTemplateParamNamesFunctionTemplateParamKindsFunctionTemplateParamTypesFunctionTemplateParamValuesFunctionTemplateParamEnablesClassDeclClassTemplateSpecKindClassTemplateParamNamesClassTemplateParamKindsClassTemplateParamTypesClassTemplateParamValuesClassTemplateParamEnablesClassCtorDeclsClassCtorParamNamesClassCtorParamTypesClassCtorParamSerializedTypes[1 1]@C[28 1]@t6@filtert42@../../../aie/aie_kernels/FirDoubleStream.hC[4 1]@t4@sin1t4@sin2t3@cint4@coutC[4 1]@t30@input_stream_cint16 * restrictt30@input_stream_cint16 * restrictt26@input_stream< cacc48_t > *t27@output_stream< cacc48_t > *C[4 1]@t37@{Q2{P{Tinput_stream{1{t{Scint16}}}}}}t37@{Q2{P{Tinput_stream{1{t{Scint16}}}}}}t35@{P{Tinput_stream{1{t{Scacc48_t}}}}}t36@{P{Toutput_stream{1{t{Scacc48_t}}}}}C[4 1]@t5@inputt5@inputt5@inputt6@outputC[4 1]@l0@l0@l0@l0@C[4 1]@l0@l0@l0@l0@C[4 1]@l0@l0@l0@l0@C[4 1]@l0@l0@l0@l1@t281@namespace DoubleStream {
      | template < int NSamples, int ShiftAcc, bool DiscardSample, bool SwapRead > 
      | void FIR_MultiKernel_cincout::
      | filter(input_stream_cint16 * restrict sin1, input_stream_cint16 * restrict sin2, input_stream< cacc48_t > * cin, output_stream< cacc48_t > * cout);
      | }t4@nonee[0 1]@e[0 1]@e[0 1]@e[0 1]@e[0 1]@t132@namespace DoubleStream {
      | template < int NSamples, int ShiftAcc, bool DiscardSample, bool SwapRead > class FIR_MultiKernel_cincout;
      | }t8@implicitC[4 1]@t8@NSamplest8@ShiftAcct13@DiscardSamplet8@SwapReadC[4 1]@t7@nontypet7@nontypet7@nontypet7@nontypeC[4 1]@t3@intt3@intt4@boolt4@boolC[4 1]@nnnnC[4 1]@l1@l1@l1@l1@C[1 1]@t54@FIR_MultiKernel_cincout(cint16 const ( & taps ) [ 4 ])C[1 1]@C[1 1]@t4@tapsC[1 1]@C[1 1]@t23@cint16 const ( &) [ 4 ]C[1 1]@C[1 1]@t20@{R{Q1{C{Scint16}4}}}
      FunctionDecl=|
      | namespace DoubleStream {
      | template < int NSamples, int ShiftAcc, bool DiscardSample, bool SwapRead > 
      | void FIR_MultiKernel_cincout::
      | filter(input_stream_cint16 * restrict sin1, input_stream_cint16 * restrict sin2, input_stream< cacc48_t > * cin, output_stream< cacc48_t > * cout);
      | }
      ClassDeclTypeOptions=|
      | C[1 1]@t132@namespace DoubleStream {
      | template < int NSamples, int ShiftAcc, bool DiscardSample, bool SwapRead > class FIR_MultiKernel_cincout;
      | }
      ClassDecl=|
      | namespace DoubleStream {
      | template < int NSamples, int ShiftAcc, bool DiscardSample, bool SwapRead > class FIR_MultiKernel_cincout;
      | }
  filter28 : aieBasic/AIE Class Kernel  KernelAllAttrs=|  PortNames={'sin1'; 'sin2'; 'cin'; 'cout'}  PortSerializedTypes={'{Q2{P{Tinput_stream{1{t{Scint16}}}}}}'; '{Q2{P{Tinput_stream{1{t{Scint16}}}}}}'; '{P{Tinput_stream{1{t{Scacc48_t}}}}}'; '{P{Toutput_stream{1{t{Scacc48_t}}}}}'}  PortWindowSizes={0.000000000000000000e+00; 0.000000000000000000e+00; 0.000000000000000000e+00; 0.000000000000000000e+00}  PortWindowMargins={0.000000000000000000e+00; 0.000000000000000000e+00; 0.000000000000000000e+00; 0.000000000000000000e+00}  PortSynchronicities={'auto', 'auto', 'auto', 'auto'}  PortSignalSizes={0.000000000000000000e+00; 0.000000000000000000e+00; 0.000000000000000000e+00; 8.000000000000000000e+00}  ClassTemplateSpecKind=implicit  ClassTemplateParamNames={'NSamples'; 'ShiftAcc'; 'DiscardSample'; 'SwapRead'}  ClassTemplateParamKinds={'nontype'; 'nontype'; 'nontype'; 'nontype'}  ClassTemplateParamTypes={'int'; 'int'; 'bool'; 'bool'}  ClassTemplateParamValues={'512', '15', '0', '0'}  ClassCtorParamNames={'taps'}  ClassCtorParamSerializedTypes={'{R{Q1{C{Scint16}4}}}'}  ClassCtorParamValues={'[-121-233i 237-96i 1454+497i 14+121i]'}  ClassIndex=1  ClassCtorIndex=1  ClassTabVisible=on  ClassTemplateParamsVisible=on  ClassCtorDeclVisible=on  ClassCtorParamsVisible=on  FunctionTabVisible=on  FunctionDecl=|  PortAttrs={ 'input', 'sin1', 'input_stream_cint16 * restrict', '', '', '', ''; 'input', 'sin2', 'input_stream_cint16 * restrict', '', '', '', ''; 'input', 'cin', 'input_stream< cacc48_t > *', '', '', '', ''; 'output', 'cout', 'output_stream< cacc48_t > *', '', '', '', 'OUTPUT_SIZE' }  PortAttrsEnables={'off', 'off', 'off', 'off', 'off', 'off', 'off';'off', 'off', 'off', 'off', 'off', 'off', 'off';'off', 'off', 'off', 'off', 'off', 'off', 'off';'off', 'off', 'off', 'off', 'off', 'off', 'on'}  SampleTime=-1  ClassDeclTypeOptions=|  ClassDecl=|  ClassTemplateParams={ 'NSamples', 'int', 'BURST_LENGTH'; 'ShiftAcc', 'int', 'SHIFT_ACC'; 'DiscardSample', 'bool', 'FALSE'; 'SwapRead', 'bool', 'FALSE' }  ClassTemplateParamsEnables={'off', 'off', 'on';'off', 'off', 'on';'off', 'off', 'on';'off', 'off', 'on'}  ClassCtorDeclTypeOptions=C[1 1]@t54@FIR_MultiKernel_cincout(cint16 const ( & taps ) [ 4 ])  ClassCtorDecl=FIR_MultiKernel_cincout(cint16 const ( & taps ) [ 4 ])  ClassCtorParams={ 'taps', 'cint16 const ( &) [ 4 ]', 'phi_4' }  KernelHeaderFile=FirDoubleStream.h  KernelClassName=DoubleStream::FIR_MultiKernel_cincout  KernelFunction=filter  KernelSourceFile=FirDoubleStream.cpp  KernelSearchPaths={'$SRC/aie_kernels'}  PreProcOptions={}  blockJsonConstraints="{\"type\":\"constraint\",\"constraintType\":\"location_kernel\",\"sid\":\"810\",\"lhs\":{\"type\":\"location\",\"templParam\":\"kernel\",\"args\":{\"type\":\"kernel\",\"name\":\"DualStreamSSR/SSR8/filter28\",\"sid\":\"810\"}},\"rhs\":{\"type\":\"tile\",\"args\":[{\"type\":\"evaluable\",\"expr\":\"29\",\"value\":29},{\"type\":\"evaluable\",\"expr\":\"2\",\"value\":2}]},\"equality\":true}"
      KernelAllAttrs=|
      | s[12;12;9;9;19;14;21;23;24;21;12;24;26;26;26;27;28;9;21;23;23;23;24;25;14;19;19;29]@FunctionNameDeclFileNamePortNamesPortTypesPortSerializedTypesPortDirectionsPortWindowSizeEnablesPortWindowMarginEnablesPortSynchronicityEnablesPortSignalSizeEnablesFunctionDeclFunctionTemplateSpecKindFunctionTemplateParamNamesFunctionTemplateParamKindsFunctionTemplateParamTypesFunctionTemplateParamValuesFunctionTemplateParamEnablesClassDeclClassTemplateSpecKindClassTemplateParamNamesClassTemplateParamKindsClassTemplateParamTypesClassTemplateParamValuesClassTemplateParamEnablesClassCtorDeclsClassCtorParamNamesClassCtorParamTypesClassCtorParamSerializedTypes[1 1]@C[28 1]@t6@filtert42@../../../aie/aie_kernels/FirDoubleStream.hC[4 1]@t4@sin1t4@sin2t3@cint4@coutC[4 1]@t30@input_stream_cint16 * restrictt30@input_stream_cint16 * restrictt26@input_stream< cacc48_t > *t27@output_stream< cacc48_t > *C[4 1]@t37@{Q2{P{Tinput_stream{1{t{Scint16}}}}}}t37@{Q2{P{Tinput_stream{1{t{Scint16}}}}}}t35@{P{Tinput_stream{1{t{Scacc48_t}}}}}t36@{P{Toutput_stream{1{t{Scacc48_t}}}}}C[4 1]@t5@inputt5@inputt5@inputt6@outputC[4 1]@l0@l0@l0@l0@C[4 1]@l0@l0@l0@l0@C[4 1]@l0@l0@l0@l0@C[4 1]@l0@l0@l0@l1@t281@namespace DoubleStream {
      | template < int NSamples, int ShiftAcc, bool DiscardSample, bool SwapRead > 
      | void FIR_MultiKernel_cincout::
      | filter(input_stream_cint16 * restrict sin1, input_stream_cint16 * restrict sin2, input_stream< cacc48_t > * cin, output_stream< cacc48_t > * cout);
      | }t4@nonee[0 1]@e[0 1]@e[0 1]@e[0 1]@e[0 1]@t132@namespace DoubleStream {
      | template < int NSamples, int ShiftAcc, bool DiscardSample, bool SwapRead > class FIR_MultiKernel_cincout;
      | }t8@implicitC[4 1]@t8@NSamplest8@ShiftAcct13@DiscardSamplet8@SwapReadC[4 1]@t7@nontypet7@nontypet7@nontypet7@nontypeC[4 1]@t3@intt3@intt4@boolt4@boolC[4 1]@nnnnC[4 1]@l1@l1@l1@l1@C[1 1]@t54@FIR_MultiKernel_cincout(cint16 const ( & taps ) [ 4 ])C[1 1]@C[1 1]@t4@tapsC[1 1]@C[1 1]@t23@cint16 const ( &) [ 4 ]C[1 1]@C[1 1]@t20@{R{Q1{C{Scint16}4}}}
      FunctionDecl=|
      | namespace DoubleStream {
      | template < int NSamples, int ShiftAcc, bool DiscardSample, bool SwapRead > 
      | void FIR_MultiKernel_cincout::
      | filter(input_stream_cint16 * restrict sin1, input_stream_cint16 * restrict sin2, input_stream< cacc48_t > * cin, output_stream< cacc48_t > * cout);
      | }
      ClassDeclTypeOptions=|
      | C[1 1]@t132@namespace DoubleStream {
      | template < int NSamples, int ShiftAcc, bool DiscardSample, bool SwapRead > class FIR_MultiKernel_cincout;
      | }
      ClassDecl=|
      | namespace DoubleStream {
      | template < int NSamples, int ShiftAcc, bool DiscardSample, bool SwapRead > class FIR_MultiKernel_cincout;
      | }
  filter29 : aieBasic/AIE Class Kernel  KernelAllAttrs=|  PortNames={'sin1'; 'sin2'; 'cin'; 'sout1'; 'sout2'}  PortSerializedTypes={'{Q2{P{Tinput_stream{1{t{Scint16}}}}}}'; '{Q2{P{Tinput_stream{1{t{Scint16}}}}}}'; '{P{Tinput_stream{1{t{Scacc48_t}}}}}'; '{Q2{P{Toutput_stream{1{t{Scint16}}}}}}'; '{Q2{P{Toutput_stream{1{t{Scint16}}}}}}'}  PortWindowSizes={0.000000000000000000e+00; 0.000000000000000000e+00; 0.000000000000000000e+00; 0.000000000000000000e+00; 0.000000000000000000e+00}  PortWindowMargins={0.000000000000000000e+00; 0.000000000000000000e+00; 0.000000000000000000e+00; 0.000000000000000000e+00; 0.000000000000000000e+00}  PortSynchronicities={'auto', 'auto', 'auto', 'auto', 'auto'}  PortSignalSizes={0.000000000000000000e+00; 0.000000000000000000e+00; 0.000000000000000000e+00; 4.000000000000000000e+00; 4.000000000000000000e+00}  ClassTemplateSpecKind=implicit  ClassTemplateParamNames={'NSamples'; 'ShiftAcc'; 'DiscardSample'; 'SwapRead'}  ClassTemplateParamKinds={'nontype'; 'nontype'; 'nontype'; 'nontype'}  ClassTemplateParamTypes={'int'; 'int'; 'bool'; 'bool'}  ClassTemplateParamValues={'512', '15', '0', '0'}  ClassCtorParamNames={'taps'}  ClassCtorParamSerializedTypes={'{R{Q1{C{Scint16}4}}}'}  ClassCtorParamValues={'[-160-111i 248+2878i 1183-239i -21-26i]'}  ClassIndex=1  ClassCtorIndex=1  ClassTabVisible=on  ClassTemplateParamsVisible=on  ClassCtorDeclVisible=on  ClassCtorParamsVisible=on  FunctionTabVisible=on  FunctionDecl=|  PortAttrs={ 'input', 'sin1', 'input_stream_cint16 * restrict', '', '', '', ''; 'input', 'sin2', 'input_stream_cint16 * restrict', '', '', '', ''; 'input', 'cin', 'input_stream< cacc48_t > *', '', '', '', ''; 'output', 'sout1', 'output_stream_cint16 * restrict', '', '', '', 'OUTPUT_SIZE/2'; 'output', 'sout2', 'output_stream_cint16 * restrict', '', '', '', 'OUTPUT_SIZE/2' }  PortAttrsEnables={'off', 'off', 'off', 'off', 'off', 'off', 'off';'off', 'off', 'off', 'off', 'off', 'off', 'off';'off', 'off', 'off', 'off', 'off', 'off', 'off';'off', 'off', 'off', 'off', 'off', 'off', 'on';'off', 'off', 'off', 'off', 'off', 'off', 'on'}  SampleTime=-1  ClassDeclTypeOptions=|  ClassDecl=|  ClassTemplateParams={ 'NSamples', 'int', 'BURST_LENGTH'; 'ShiftAcc', 'int', 'SHIFT_ACC'; 'DiscardSample', 'bool', 'FALSE'; 'SwapRead', 'bool', 'FALSE' }  ClassTemplateParamsEnables={'off', 'off', 'on';'off', 'off', 'on';'off', 'off', 'on';'off', 'off', 'on'}  ClassCtorDeclTypeOptions=C[1 1]@t50@FIR_MultiKernel_cin(cint16 const ( & taps ) [ 4 ])  ClassCtorDecl=FIR_MultiKernel_cin(cint16 const ( & taps ) [ 4 ])  ClassCtorParams={ 'taps', 'cint16 const ( &) [ 4 ]', 'phi_5' }  KernelHeaderFile=FirDoubleStream.h  KernelClassName=DoubleStream::FIR_MultiKernel_cin  KernelFunction=filter  KernelSourceFile=FirDoubleStream.cpp  KernelSearchPaths={'$SRC/aie_kernels'}  PreProcOptions={}  blockJsonConstraints="{\"type\":\"constraint\",\"constraintType\":\"location_kernel\",\"sid\":\"811\",\"lhs\":{\"type\":\"location\",\"templParam\":\"kernel\",\"args\":{\"type\":\"kernel\",\"name\":\"DualStreamSSR/SSR8/filter29\",\"sid\":\"811\"}},\"rhs\":{\"type\":\"tile\",\"args\":[{\"type\":\"evaluable\",\"expr\":\"30\",\"value\":30},{\"type\":\"evaluable\",\"expr\":\"2\",\"value\":2}]},\"equality\":true}"
      KernelAllAttrs=|
      | s[12;12;9;9;19;14;21;23;24;21;12;24;26;26;26;27;28;9;21;23;23;23;24;25;14;19;19;29]@FunctionNameDeclFileNamePortNamesPortTypesPortSerializedTypesPortDirectionsPortWindowSizeEnablesPortWindowMarginEnablesPortSynchronicityEnablesPortSignalSizeEnablesFunctionDeclFunctionTemplateSpecKindFunctionTemplateParamNamesFunctionTemplateParamKindsFunctionTemplateParamTypesFunctionTemplateParamValuesFunctionTemplateParamEnablesClassDeclClassTemplateSpecKindClassTemplateParamNamesClassTemplateParamKindsClassTemplateParamTypesClassTemplateParamValuesClassTemplateParamEnablesClassCtorDeclsClassCtorParamNamesClassCtorParamTypesClassCtorParamSerializedTypes[1 1]@C[28 1]@t6@filtert42@../../../aie/aie_kernels/FirDoubleStream.hC[5 1]@t4@sin1t4@sin2t3@cint5@sout1t5@sout2C[5 1]@t30@input_stream_cint16 * restrictt30@input_stream_cint16 * restrictt26@input_stream< cacc48_t > *t31@output_stream_cint16 * restrictt31@output_stream_cint16 * restrictC[5 1]@t37@{Q2{P{Tinput_stream{1{t{Scint16}}}}}}t37@{Q2{P{Tinput_stream{1{t{Scint16}}}}}}t35@{P{Tinput_stream{1{t{Scacc48_t}}}}}t38@{Q2{P{Toutput_stream{1{t{Scint16}}}}}}t38@{Q2{P{Toutput_stream{1{t{Scint16}}}}}}C[5 1]@t5@inputt5@inputt5@inputt6@outputt6@outputC[5 1]@l0@l0@l0@l0@l0@C[5 1]@l0@l0@l0@l0@l0@C[5 1]@l0@l0@l0@l0@l0@C[5 1]@l0@l0@l0@l1@l1@t321@namespace DoubleStream {
      | template < int NSamples, int ShiftAcc, bool DiscardSample, bool SwapRead > 
      | void FIR_MultiKernel_cin::
      | filter(input_stream_cint16 * restrict sin1, input_stream_cint16 * restrict sin2, input_stream< cacc48_t > * cin, output_stream_cint16 * restrict sout1, output_stream_cint16 * restrict sout2);
      | }t4@nonee[0 1]@e[0 1]@e[0 1]@e[0 1]@e[0 1]@t128@namespace DoubleStream {
      | template < int NSamples, int ShiftAcc, bool DiscardSample, bool SwapRead > class FIR_MultiKernel_cin;
      | }t8@implicitC[4 1]@t8@NSamplest8@ShiftAcct13@DiscardSamplet8@SwapReadC[4 1]@t7@nontypet7@nontypet7@nontypet7@nontypeC[4 1]@t3@intt3@intt4@boolt4@boolC[4 1]@nnnnC[4 1]@l1@l1@l1@l1@C[1 1]@t50@FIR_MultiKernel_cin(cint16 const ( & taps ) [ 4 ])C[1 1]@C[1 1]@t4@tapsC[1 1]@C[1 1]@t23@cint16 const ( &) [ 4 ]C[1 1]@C[1 1]@t20@{R{Q1{C{Scint16}4}}}
      FunctionDecl=|
      | namespace DoubleStream {
      | template < int NSamples, int ShiftAcc, bool DiscardSample, bool SwapRead > 
      | void FIR_MultiKernel_cin::
      | filter(input_stream_cint16 * restrict sin1, input_stream_cint16 * restrict sin2, input_stream< cacc48_t > * cin, output_stream_cint16 * restrict sout1, output_stream_cint16 * restrict sout2);
      | }
      ClassDeclTypeOptions=|
      | C[1 1]@t128@namespace DoubleStream {
      | template < int NSamples, int ShiftAcc, bool DiscardSample, bool SwapRead > class FIR_MultiKernel_cin;
      | }
      ClassDecl=|
      | namespace DoubleStream {
      | template < int NSamples, int ShiftAcc, bool DiscardSample, bool SwapRead > class FIR_MultiKernel_cin;
      | }
  filter3 : aieBasic/AIE Class Kernel  KernelAllAttrs=|  PortNames={'sin1'; 'sin2'; 'cin'; 'cout'}  PortSerializedTypes={'{Q2{P{Tinput_stream{1{t{Scint16}}}}}}'; '{Q2{P{Tinput_stream{1{t{Scint16}}}}}}'; '{P{Tinput_stream{1{t{Scacc48_t}}}}}'; '{P{Toutput_stream{1{t{Scacc48_t}}}}}'}  PortWindowSizes={0.000000000000000000e+00; 0.000000000000000000e+00; 0.000000000000000000e+00; 0.000000000000000000e+00}  PortWindowMargins={0.000000000000000000e+00; 0.000000000000000000e+00; 0.000000000000000000e+00; 0.000000000000000000e+00}  PortSynchronicities={'auto', 'auto', 'auto', 'auto'}  PortSignalSizes={0.000000000000000000e+00; 0.000000000000000000e+00; 0.000000000000000000e+00; 8.000000000000000000e+00}  ClassTemplateSpecKind=implicit  ClassTemplateParamNames={'NSamples'; 'ShiftAcc'; 'DiscardSample'; 'SwapRead'}  ClassTemplateParamKinds={'nontype'; 'nontype'; 'nontype'; 'nontype'}  ClassTemplateParamTypes={'int'; 'int'; 'bool'; 'bool'}  ClassTemplateParamValues={'512', '15', '0', '0'}  ClassCtorParamNames={'taps'}  ClassCtorParamSerializedTypes={'{R{Q1{C{Scint16}4}}}'}  ClassCtorParamValues={'[14-121i 1454-497i 237+96i -121+233i]'}  ClassIndex=1  ClassCtorIndex=1  ClassTabVisible=on  ClassTemplateParamsVisible=on  ClassCtorDeclVisible=on  ClassCtorParamsVisible=on  FunctionTabVisible=on  FunctionDecl=|  PortAttrs={ 'input', 'sin1', 'input_stream_cint16 * restrict', '', '', '', ''; 'input', 'sin2', 'input_stream_cint16 * restrict', '', '', '', ''; 'input', 'cin', 'input_stream< cacc48_t > *', '', '', '', ''; 'output', 'cout', 'output_stream< cacc48_t > *', '', '', '', 'OUTPUT_SIZE' }  PortAttrsEnables={'off', 'off', 'off', 'off', 'off', 'off', 'off';'off', 'off', 'off', 'off', 'off', 'off', 'off';'off', 'off', 'off', 'off', 'off', 'off', 'off';'off', 'off', 'off', 'off', 'off', 'off', 'on'}  SampleTime=-1  ClassDeclTypeOptions=|  ClassDecl=|  ClassTemplateParams={ 'NSamples', 'int', 'BURST_LENGTH'; 'ShiftAcc', 'int', 'SHIFT_ACC'; 'DiscardSample', 'bool', 'FALSE'; 'SwapRead', 'bool', 'FALSE' }  ClassTemplateParamsEnables={'off', 'off', 'on';'off', 'off', 'on';'off', 'off', 'on';'off', 'off', 'on'}  ClassCtorDeclTypeOptions=C[1 1]@t54@FIR_MultiKernel_cincout(cint16 const ( & taps ) [ 4 ])  ClassCtorDecl=FIR_MultiKernel_cincout(cint16 const ( & taps ) [ 4 ])  ClassCtorParams={ 'taps', 'cint16 const ( &) [ 4 ]', 'phi_3' }  KernelHeaderFile=FirDoubleStream.h  KernelClassName=DoubleStream::FIR_MultiKernel_cincout  KernelFunction=filter  KernelSourceFile=FirDoubleStream.cpp  KernelSearchPaths={'$SRC/aie_kernels'}  PreProcOptions={}  blockJsonConstraints="{\"type\":\"constraint\",\"constraintType\":\"location_kernel\",\"sid\":\"812\",\"lhs\":{\"type\":\"location\",\"templParam\":\"kernel\",\"args\":{\"type\":\"kernel\",\"name\":\"DualStreamSSR/SSR8/filter3\",\"sid\":\"812\"}},\"rhs\":{\"type\":\"tile\",\"args\":[{\"type\":\"evaluable\",\"expr\":\"26\",\"value\":26},{\"type\":\"evaluable\",\"expr\":\"0\",\"value\":0}]},\"equality\":true}"
      KernelAllAttrs=|
      | s[12;12;9;9;19;14;21;23;24;21;12;24;26;26;26;27;28;9;21;23;23;23;24;25;14;19;19;29]@FunctionNameDeclFileNamePortNamesPortTypesPortSerializedTypesPortDirectionsPortWindowSizeEnablesPortWindowMarginEnablesPortSynchronicityEnablesPortSignalSizeEnablesFunctionDeclFunctionTemplateSpecKindFunctionTemplateParamNamesFunctionTemplateParamKindsFunctionTemplateParamTypesFunctionTemplateParamValuesFunctionTemplateParamEnablesClassDeclClassTemplateSpecKindClassTemplateParamNamesClassTemplateParamKindsClassTemplateParamTypesClassTemplateParamValuesClassTemplateParamEnablesClassCtorDeclsClassCtorParamNamesClassCtorParamTypesClassCtorParamSerializedTypes[1 1]@C[28 1]@t6@filtert42@../../../aie/aie_kernels/FirDoubleStream.hC[4 1]@t4@sin1t4@sin2t3@cint4@coutC[4 1]@t30@input_stream_cint16 * restrictt30@input_stream_cint16 * restrictt26@input_stream< cacc48_t > *t27@output_stream< cacc48_t > *C[4 1]@t37@{Q2{P{Tinput_stream{1{t{Scint16}}}}}}t37@{Q2{P{Tinput_stream{1{t{Scint16}}}}}}t35@{P{Tinput_stream{1{t{Scacc48_t}}}}}t36@{P{Toutput_stream{1{t{Scacc48_t}}}}}C[4 1]@t5@inputt5@inputt5@inputt6@outputC[4 1]@l0@l0@l0@l0@C[4 1]@l0@l0@l0@l0@C[4 1]@l0@l0@l0@l0@C[4 1]@l0@l0@l0@l1@t281@namespace DoubleStream {
      | template < int NSamples, int ShiftAcc, bool DiscardSample, bool SwapRead > 
      | void FIR_MultiKernel_cincout::
      | filter(input_stream_cint16 * restrict sin1, input_stream_cint16 * restrict sin2, input_stream< cacc48_t > * cin, output_stream< cacc48_t > * cout);
      | }t4@nonee[0 1]@e[0 1]@e[0 1]@e[0 1]@e[0 1]@t132@namespace DoubleStream {
      | template < int NSamples, int ShiftAcc, bool DiscardSample, bool SwapRead > class FIR_MultiKernel_cincout;
      | }t8@implicitC[4 1]@t8@NSamplest8@ShiftAcct13@DiscardSamplet8@SwapReadC[4 1]@t7@nontypet7@nontypet7@nontypet7@nontypeC[4 1]@t3@intt3@intt4@boolt4@boolC[4 1]@nnnnC[4 1]@l1@l1@l1@l1@C[1 1]@t54@FIR_MultiKernel_cincout(cint16 const ( & taps ) [ 4 ])C[1 1]@C[1 1]@t4@tapsC[1 1]@C[1 1]@t23@cint16 const ( &) [ 4 ]C[1 1]@C[1 1]@t20@{R{Q1{C{Scint16}4}}}
      FunctionDecl=|
      | namespace DoubleStream {
      | template < int NSamples, int ShiftAcc, bool DiscardSample, bool SwapRead > 
      | void FIR_MultiKernel_cincout::
      | filter(input_stream_cint16 * restrict sin1, input_stream_cint16 * restrict sin2, input_stream< cacc48_t > * cin, output_stream< cacc48_t > * cout);
      | }
      ClassDeclTypeOptions=|
      | C[1 1]@t132@namespace DoubleStream {
      | template < int NSamples, int ShiftAcc, bool DiscardSample, bool SwapRead > class FIR_MultiKernel_cincout;
      | }
      ClassDecl=|
      | namespace DoubleStream {
      | template < int NSamples, int ShiftAcc, bool DiscardSample, bool SwapRead > class FIR_MultiKernel_cincout;
      | }
  filter30 : aieBasic/AIE Class Kernel  KernelAllAttrs=|  PortNames={'sin1'; 'sin2'; 'cout'}  PortSerializedTypes={'{Q2{P{Tinput_stream{1{t{Scint16}}}}}}'; '{Q2{P{Tinput_stream{1{t{Scint16}}}}}}'; '{P{Toutput_stream{1{t{Scacc48_t}}}}}'}  PortWindowSizes={0.000000000000000000e+00; 0.000000000000000000e+00; 0.000000000000000000e+00}  PortWindowMargins={0.000000000000000000e+00; 0.000000000000000000e+00; 0.000000000000000000e+00}  PortSynchronicities={'auto', 'auto', 'auto'}  PortSignalSizes={0.000000000000000000e+00; 0.000000000000000000e+00; 8.000000000000000000e+00}  ClassTemplateSpecKind=implicit  ClassTemplateParamNames={'NSamples'; 'ShiftAcc'; 'DiscardSample'; 'SwapRead'}  ClassTemplateParamKinds={'nontype'; 'nontype'; 'nontype'; 'nontype'}  ClassTemplateParamTypes={'int'; 'int'; 'bool'; 'bool'}  ClassTemplateParamValues={'512', '15', '0', '0'}  ClassCtorParamNames={'taps'}  ClassCtorParamSerializedTypes={'{R{Q1{C{Scint16}4}}}'}  ClassCtorParamValues={'[-121-233i 237-96i 1454+497i 14+121i]'}  ClassIndex=1  ClassCtorIndex=1  ClassTabVisible=on  ClassTemplateParamsVisible=on  ClassCtorDeclVisible=on  ClassCtorParamsVisible=on  FunctionTabVisible=on  FunctionDecl=|  PortAttrs={ 'input', 'sin1', 'input_stream_cint16 * restrict', '', '', '', ''; 'input', 'sin2', 'input_stream_cint16 * restrict', '', '', '', ''; 'output', 'cout', 'output_stream< cacc48_t > *', '', '', '', 'OUTPUT_SIZE' }  PortAttrsEnables={'off', 'off', 'off', 'off', 'off', 'off', 'off';'off', 'off', 'off', 'off', 'off', 'off', 'off';'off', 'off', 'off', 'off', 'off', 'off', 'on'}  SampleTime=-1  ClassDeclTypeOptions=|  ClassDecl=|  ClassTemplateParams={ 'NSamples', 'int', 'BURST_LENGTH'; 'ShiftAcc', 'int', 'SHIFT_ACC'; 'DiscardSample', 'bool', 'FALSE'; 'SwapRead', 'bool', 'FALSE' }  ClassTemplateParamsEnables={'off', 'off', 'on';'off', 'off', 'on';'off', 'off', 'on';'off', 'off', 'on'}  ClassCtorDeclTypeOptions=C[1 1]@t51@FIR_MultiKernel_cout(cint16 const ( & taps ) [ 4 ])  ClassCtorDecl=FIR_MultiKernel_cout(cint16 const ( & taps ) [ 4 ])  ClassCtorParams={ 'taps', 'cint16 const ( &) [ 4 ]', 'phi_4' }  KernelHeaderFile=FirDoubleStream.h  KernelClassName=DoubleStream::FIR_MultiKernel_cout  KernelFunction=filter  KernelSourceFile=FirDoubleStream.cpp  KernelSearchPaths={'$SRC/aie_kernels'}  PreProcOptions={}  blockJsonConstraints="{\"type\":\"constraint\",\"constraintType\":\"location_kernel\",\"sid\":\"813\",\"lhs\":{\"type\":\"location\",\"templParam\":\"kernel\",\"args\":{\"type\":\"kernel\",\"name\":\"DualStreamSSR/SSR8/filter30\",\"sid\":\"813\"}},\"rhs\":{\"type\":\"tile\",\"args\":[{\"type\":\"evaluable\",\"expr\":\"30\",\"value\":30},{\"type\":\"evaluable\",\"expr\":\"3\",\"value\":3}]},\"equality\":true}"
      KernelAllAttrs=|
      | s[12;12;9;9;19;14;21;23;24;21;12;24;26;26;26;27;28;9;21;23;23;23;24;25;14;19;19;29]@FunctionNameDeclFileNamePortNamesPortTypesPortSerializedTypesPortDirectionsPortWindowSizeEnablesPortWindowMarginEnablesPortSynchronicityEnablesPortSignalSizeEnablesFunctionDeclFunctionTemplateSpecKindFunctionTemplateParamNamesFunctionTemplateParamKindsFunctionTemplateParamTypesFunctionTemplateParamValuesFunctionTemplateParamEnablesClassDeclClassTemplateSpecKindClassTemplateParamNamesClassTemplateParamKindsClassTemplateParamTypesClassTemplateParamValuesClassTemplateParamEnablesClassCtorDeclsClassCtorParamNamesClassCtorParamTypesClassCtorParamSerializedTypes[1 1]@C[28 1]@t6@filtert42@../../../aie/aie_kernels/FirDoubleStream.hC[3 1]@t4@sin1t4@sin2t4@coutC[3 1]@t30@input_stream_cint16 * restrictt30@input_stream_cint16 * restrictt27@output_stream< cacc48_t > *C[3 1]@t37@{Q2{P{Tinput_stream{1{t{Scint16}}}}}}t37@{Q2{P{Tinput_stream{1{t{Scint16}}}}}}t36@{P{Toutput_stream{1{t{Scacc48_t}}}}}C[3 1]@t5@inputt5@inputt6@outputC[3 1]@l0@l0@l0@C[3 1]@l0@l0@l0@C[3 1]@l0@l0@l0@C[3 1]@l0@l0@l1@t246@namespace DoubleStream {
      | template < int NSamples, int ShiftAcc, bool DiscardSample, bool SwapRead > 
      | void FIR_MultiKernel_cout::
      | filter(input_stream_cint16 * restrict sin1, input_stream_cint16 * restrict sin2, output_stream< cacc48_t > * cout);
      | }t4@nonee[0 1]@e[0 1]@e[0 1]@e[0 1]@e[0 1]@t129@namespace DoubleStream {
      | template < int NSamples, int ShiftAcc, bool DiscardSample, bool SwapRead > class FIR_MultiKernel_cout;
      | }t8@implicitC[4 1]@t8@NSamplest8@ShiftAcct13@DiscardSamplet8@SwapReadC[4 1]@t7@nontypet7@nontypet7@nontypet7@nontypeC[4 1]@t3@intt3@intt4@boolt4@boolC[4 1]@nnnnC[4 1]@l1@l1@l1@l1@C[1 1]@t51@FIR_MultiKernel_cout(cint16 const ( & taps ) [ 4 ])C[1 1]@C[1 1]@t4@tapsC[1 1]@C[1 1]@t23@cint16 const ( &) [ 4 ]C[1 1]@C[1 1]@t20@{R{Q1{C{Scint16}4}}}
      FunctionDecl=|
      | namespace DoubleStream {
      | template < int NSamples, int ShiftAcc, bool DiscardSample, bool SwapRead > 
      | void FIR_MultiKernel_cout::
      | filter(input_stream_cint16 * restrict sin1, input_stream_cint16 * restrict sin2, output_stream< cacc48_t > * cout);
      | }
      ClassDeclTypeOptions=|
      | C[1 1]@t129@namespace DoubleStream {
      | template < int NSamples, int ShiftAcc, bool DiscardSample, bool SwapRead > class FIR_MultiKernel_cout;
      | }
      ClassDecl=|
      | namespace DoubleStream {
      | template < int NSamples, int ShiftAcc, bool DiscardSample, bool SwapRead > class FIR_MultiKernel_cout;
      | }
  filter31 : aieBasic/AIE Class Kernel  KernelAllAttrs=|  PortNames={'sin1'; 'sin2'; 'cin'; 'cout'}  PortSerializedTypes={'{Q2{P{Tinput_stream{1{t{Scint16}}}}}}'; '{Q2{P{Tinput_stream{1{t{Scint16}}}}}}'; '{P{Tinput_stream{1{t{Scacc48_t}}}}}'; '{P{Toutput_stream{1{t{Scacc48_t}}}}}'}  PortWindowSizes={0.000000000000000000e+00; 0.000000000000000000e+00; 0.000000000000000000e+00; 0.000000000000000000e+00}  PortWindowMargins={0.000000000000000000e+00; 0.000000000000000000e+00; 0.000000000000000000e+00; 0.000000000000000000e+00}  PortSynchronicities={'auto', 'auto', 'auto', 'auto'}  PortSignalSizes={0.000000000000000000e+00; 0.000000000000000000e+00; 0.000000000000000000e+00; 8.000000000000000000e+00}  ClassTemplateSpecKind=implicit  ClassTemplateParamNames={'NSamples'; 'ShiftAcc'; 'DiscardSample'; 'SwapRead'}  ClassTemplateParamKinds={'nontype'; 'nontype'; 'nontype'; 'nontype'}  ClassTemplateParamTypes={'int'; 'int'; 'bool'; 'bool'}  ClassTemplateParamValues={'512', '15', '0', '0'}  ClassCtorParamNames={'taps'}  ClassCtorParamSerializedTypes={'{R{Q1{C{Scint16}4}}}'}  ClassCtorParamValues={'[14-121i 1454-497i 237+96i -121+233i]'}  ClassIndex=1  ClassCtorIndex=1  ClassTabVisible=on  ClassTemplateParamsVisible=on  ClassCtorDeclVisible=on  ClassCtorParamsVisible=on  FunctionTabVisible=on  FunctionDecl=|  PortAttrs={ 'input', 'sin1', 'input_stream_cint16 * restrict', '', '', '', ''; 'input', 'sin2', 'input_stream_cint16 * restrict', '', '', '', ''; 'input', 'cin', 'input_stream< cacc48_t > *', '', '', '', ''; 'output', 'cout', 'output_stream< cacc48_t > *', '', '', '', 'OUTPUT_SIZE' }  PortAttrsEnables={'off', 'off', 'off', 'off', 'off', 'off', 'off';'off', 'off', 'off', 'off', 'off', 'off', 'off';'off', 'off', 'off', 'off', 'off', 'off', 'off';'off', 'off', 'off', 'off', 'off', 'off', 'on'}  SampleTime=-1  ClassDeclTypeOptions=|  ClassDecl=|  ClassTemplateParams={ 'NSamples', 'int', 'BURST_LENGTH'; 'ShiftAcc', 'int', 'SHIFT_ACC'; 'DiscardSample', 'bool', 'FALSE'; 'SwapRead', 'bool', 'FALSE' }  ClassTemplateParamsEnables={'off', 'off', 'on';'off', 'off', 'on';'off', 'off', 'on';'off', 'off', 'on'}  ClassCtorDeclTypeOptions=C[1 1]@t54@FIR_MultiKernel_cincout(cint16 const ( & taps ) [ 4 ])  ClassCtorDecl=FIR_MultiKernel_cincout(cint16 const ( & taps ) [ 4 ])  ClassCtorParams={ 'taps', 'cint16 const ( &) [ 4 ]', 'phi_3' }  KernelHeaderFile=FirDoubleStream.h  KernelClassName=DoubleStream::FIR_MultiKernel_cincout  KernelFunction=filter  KernelSourceFile=FirDoubleStream.cpp  KernelSearchPaths={'$SRC/aie_kernels'}  PreProcOptions={}  blockJsonConstraints="{\"type\":\"constraint\",\"constraintType\":\"location_kernel\",\"sid\":\"814\",\"lhs\":{\"type\":\"location\",\"templParam\":\"kernel\",\"args\":{\"type\":\"kernel\",\"name\":\"DualStreamSSR/SSR8/filter31\",\"sid\":\"814\"}},\"rhs\":{\"type\":\"tile\",\"args\":[{\"type\":\"evaluable\",\"expr\":\"29\",\"value\":29},{\"type\":\"evaluable\",\"expr\":\"3\",\"value\":3}]},\"equality\":true}"
      KernelAllAttrs=|
      | s[12;12;9;9;19;14;21;23;24;21;12;24;26;26;26;27;28;9;21;23;23;23;24;25;14;19;19;29]@FunctionNameDeclFileNamePortNamesPortTypesPortSerializedTypesPortDirectionsPortWindowSizeEnablesPortWindowMarginEnablesPortSynchronicityEnablesPortSignalSizeEnablesFunctionDeclFunctionTemplateSpecKindFunctionTemplateParamNamesFunctionTemplateParamKindsFunctionTemplateParamTypesFunctionTemplateParamValuesFunctionTemplateParamEnablesClassDeclClassTemplateSpecKindClassTemplateParamNamesClassTemplateParamKindsClassTemplateParamTypesClassTemplateParamValuesClassTemplateParamEnablesClassCtorDeclsClassCtorParamNamesClassCtorParamTypesClassCtorParamSerializedTypes[1 1]@C[28 1]@t6@filtert42@../../../aie/aie_kernels/FirDoubleStream.hC[4 1]@t4@sin1t4@sin2t3@cint4@coutC[4 1]@t30@input_stream_cint16 * restrictt30@input_stream_cint16 * restrictt26@input_stream< cacc48_t > *t27@output_stream< cacc48_t > *C[4 1]@t37@{Q2{P{Tinput_stream{1{t{Scint16}}}}}}t37@{Q2{P{Tinput_stream{1{t{Scint16}}}}}}t35@{P{Tinput_stream{1{t{Scacc48_t}}}}}t36@{P{Toutput_stream{1{t{Scacc48_t}}}}}C[4 1]@t5@inputt5@inputt5@inputt6@outputC[4 1]@l0@l0@l0@l0@C[4 1]@l0@l0@l0@l0@C[4 1]@l0@l0@l0@l0@C[4 1]@l0@l0@l0@l1@t281@namespace DoubleStream {
      | template < int NSamples, int ShiftAcc, bool DiscardSample, bool SwapRead > 
      | void FIR_MultiKernel_cincout::
      | filter(input_stream_cint16 * restrict sin1, input_stream_cint16 * restrict sin2, input_stream< cacc48_t > * cin, output_stream< cacc48_t > * cout);
      | }t4@nonee[0 1]@e[0 1]@e[0 1]@e[0 1]@e[0 1]@t132@namespace DoubleStream {
      | template < int NSamples, int ShiftAcc, bool DiscardSample, bool SwapRead > class FIR_MultiKernel_cincout;
      | }t8@implicitC[4 1]@t8@NSamplest8@ShiftAcct13@DiscardSamplet8@SwapReadC[4 1]@t7@nontypet7@nontypet7@nontypet7@nontypeC[4 1]@t3@intt3@intt4@boolt4@boolC[4 1]@nnnnC[4 1]@l1@l1@l1@l1@C[1 1]@t54@FIR_MultiKernel_cincout(cint16 const ( & taps ) [ 4 ])C[1 1]@C[1 1]@t4@tapsC[1 1]@C[1 1]@t23@cint16 const ( &) [ 4 ]C[1 1]@C[1 1]@t20@{R{Q1{C{Scint16}4}}}
      FunctionDecl=|
      | namespace DoubleStream {
      | template < int NSamples, int ShiftAcc, bool DiscardSample, bool SwapRead > 
      | void FIR_MultiKernel_cincout::
      | filter(input_stream_cint16 * restrict sin1, input_stream_cint16 * restrict sin2, input_stream< cacc48_t > * cin, output_stream< cacc48_t > * cout);
      | }
      ClassDeclTypeOptions=|
      | C[1 1]@t132@namespace DoubleStream {
      | template < int NSamples, int ShiftAcc, bool DiscardSample, bool SwapRead > class FIR_MultiKernel_cincout;
      | }
      ClassDecl=|
      | namespace DoubleStream {
      | template < int NSamples, int ShiftAcc, bool DiscardSample, bool SwapRead > class FIR_MultiKernel_cincout;
      | }
  filter32 : aieBasic/AIE Class Kernel  KernelAllAttrs=|  PortNames={'sin1'; 'sin2'; 'cout'}  PortSerializedTypes={'{Q2{P{Tinput_stream{1{t{Scint16}}}}}}'; '{Q2{P{Tinput_stream{1{t{Scint16}}}}}}'; '{P{Toutput_stream{1{t{Scacc48_t}}}}}'}  PortWindowSizes={0.000000000000000000e+00; 0.000000000000000000e+00; 0.000000000000000000e+00}  PortWindowMargins={0.000000000000000000e+00; 0.000000000000000000e+00; 0.000000000000000000e+00}  PortSynchronicities={'auto', 'auto', 'auto'}  PortSignalSizes={0.000000000000000000e+00; 0.000000000000000000e+00; 8.000000000000000000e+00}  ClassTemplateSpecKind=implicit  ClassTemplateParamNames={'NSamples'; 'ShiftAcc'; 'DiscardSample'; 'SwapRead'}  ClassTemplateParamKinds={'nontype'; 'nontype'; 'nontype'; 'nontype'}  ClassTemplateParamTypes={'int'; 'int'; 'bool'; 'bool'}  ClassTemplateParamValues={'512', '15', '1', '0'}  ClassCtorParamNames={'taps'}  ClassCtorParamSerializedTypes={'{R{Q1{C{Scint16}4}}}'}  ClassCtorParamValues={'[-121-233i 237-96i 1454+497i 14+121i]'}  ClassIndex=1  ClassCtorIndex=1  ClassTabVisible=on  ClassTemplateParamsVisible=on  ClassCtorDeclVisible=on  ClassCtorParamsVisible=on  FunctionTabVisible=on  FunctionDecl=|  PortAttrs={ 'input', 'sin1', 'input_stream_cint16 * restrict', '', '', '', ''; 'input', 'sin2', 'input_stream_cint16 * restrict', '', '', '', ''; 'output', 'cout', 'output_stream< cacc48_t > *', '', '', '', 'OUTPUT_SIZE' }  PortAttrsEnables={'off', 'off', 'off', 'off', 'off', 'off', 'off';'off', 'off', 'off', 'off', 'off', 'off', 'off';'off', 'off', 'off', 'off', 'off', 'off', 'on'}  SampleTime=-1  ClassDeclTypeOptions=|  ClassDecl=|  ClassTemplateParams={ 'NSamples', 'int', 'BURST_LENGTH'; 'ShiftAcc', 'int', 'SHIFT_ACC'; 'DiscardSample', 'bool', 'TRUE'; 'SwapRead', 'bool', 'FALSE' }  ClassTemplateParamsEnables={'off', 'off', 'on';'off', 'off', 'on';'off', 'off', 'on';'off', 'off', 'on'}  ClassCtorDeclTypeOptions=C[1 1]@t51@FIR_MultiKernel_cout(cint16 const ( & taps ) [ 4 ])  ClassCtorDecl=FIR_MultiKernel_cout(cint16 const ( & taps ) [ 4 ])  ClassCtorParams={ 'taps', 'cint16 const ( &) [ 4 ]', 'phi_4' }  KernelHeaderFile=FirDoubleStream.h  KernelClassName=DoubleStream::FIR_MultiKernel_cout  KernelFunction=filter  KernelSourceFile=FirDoubleStream.cpp  KernelSearchPaths={'$SRC/aie_kernels'}  PreProcOptions={}  blockJsonConstraints="{\"type\":\"constraint\",\"constraintType\":\"location_kernel\",\"sid\":\"815\",\"lhs\":{\"type\":\"location\",\"templParam\":\"kernel\",\"args\":{\"type\":\"kernel\",\"name\":\"DualStreamSSR/SSR8/filter32\",\"sid\":\"815\"}},\"rhs\":{\"type\":\"tile\",\"args\":[{\"type\":\"evaluable\",\"expr\":\"23\",\"value\":23},{\"type\":\"evaluable\",\"expr\":\"4\",\"value\":4}]},\"equality\":true}"
      KernelAllAttrs=|
      | s[12;12;9;9;19;14;21;23;24;21;12;24;26;26;26;27;28;9;21;23;23;23;24;25;14;19;19;29]@FunctionNameDeclFileNamePortNamesPortTypesPortSerializedTypesPortDirectionsPortWindowSizeEnablesPortWindowMarginEnablesPortSynchronicityEnablesPortSignalSizeEnablesFunctionDeclFunctionTemplateSpecKindFunctionTemplateParamNamesFunctionTemplateParamKindsFunctionTemplateParamTypesFunctionTemplateParamValuesFunctionTemplateParamEnablesClassDeclClassTemplateSpecKindClassTemplateParamNamesClassTemplateParamKindsClassTemplateParamTypesClassTemplateParamValuesClassTemplateParamEnablesClassCtorDeclsClassCtorParamNamesClassCtorParamTypesClassCtorParamSerializedTypes[1 1]@C[28 1]@t6@filtert42@../../../aie/aie_kernels/FirDoubleStream.hC[3 1]@t4@sin1t4@sin2t4@coutC[3 1]@t30@input_stream_cint16 * restrictt30@input_stream_cint16 * restrictt27@output_stream< cacc48_t > *C[3 1]@t37@{Q2{P{Tinput_stream{1{t{Scint16}}}}}}t37@{Q2{P{Tinput_stream{1{t{Scint16}}}}}}t36@{P{Toutput_stream{1{t{Scacc48_t}}}}}C[3 1]@t5@inputt5@inputt6@outputC[3 1]@l0@l0@l0@C[3 1]@l0@l0@l0@C[3 1]@l0@l0@l0@C[3 1]@l0@l0@l1@t246@namespace DoubleStream {
      | template < int NSamples, int ShiftAcc, bool DiscardSample, bool SwapRead > 
      | void FIR_MultiKernel_cout::
      | filter(input_stream_cint16 * restrict sin1, input_stream_cint16 * restrict sin2, output_stream< cacc48_t > * cout);
      | }t4@nonee[0 1]@e[0 1]@e[0 1]@e[0 1]@e[0 1]@t129@namespace DoubleStream {
      | template < int NSamples, int ShiftAcc, bool DiscardSample, bool SwapRead > class FIR_MultiKernel_cout;
      | }t8@implicitC[4 1]@t8@NSamplest8@ShiftAcct13@DiscardSamplet8@SwapReadC[4 1]@t7@nontypet7@nontypet7@nontypet7@nontypeC[4 1]@t3@intt3@intt4@boolt4@boolC[4 1]@nnnnC[4 1]@l1@l1@l1@l1@C[1 1]@t51@FIR_MultiKernel_cout(cint16 const ( & taps ) [ 4 ])C[1 1]@C[1 1]@t4@tapsC[1 1]@C[1 1]@t23@cint16 const ( &) [ 4 ]C[1 1]@C[1 1]@t20@{R{Q1{C{Scint16}4}}}
      FunctionDecl=|
      | namespace DoubleStream {
      | template < int NSamples, int ShiftAcc, bool DiscardSample, bool SwapRead > 
      | void FIR_MultiKernel_cout::
      | filter(input_stream_cint16 * restrict sin1, input_stream_cint16 * restrict sin2, output_stream< cacc48_t > * cout);
      | }
      ClassDeclTypeOptions=|
      | C[1 1]@t129@namespace DoubleStream {
      | template < int NSamples, int ShiftAcc, bool DiscardSample, bool SwapRead > class FIR_MultiKernel_cout;
      | }
      ClassDecl=|
      | namespace DoubleStream {
      | template < int NSamples, int ShiftAcc, bool DiscardSample, bool SwapRead > class FIR_MultiKernel_cout;
      | }
  filter33 : aieBasic/AIE Class Kernel  KernelAllAttrs=|  PortNames={'sin1'; 'sin2'; 'cin'; 'cout'}  PortSerializedTypes={'{Q2{P{Tinput_stream{1{t{Scint16}}}}}}'; '{Q2{P{Tinput_stream{1{t{Scint16}}}}}}'; '{P{Tinput_stream{1{t{Scacc48_t}}}}}'; '{P{Toutput_stream{1{t{Scacc48_t}}}}}'}  PortWindowSizes={0.000000000000000000e+00; 0.000000000000000000e+00; 0.000000000000000000e+00; 0.000000000000000000e+00}  PortWindowMargins={0.000000000000000000e+00; 0.000000000000000000e+00; 0.000000000000000000e+00; 0.000000000000000000e+00}  PortSynchronicities={'auto', 'auto', 'auto', 'auto'}  PortSignalSizes={0.000000000000000000e+00; 0.000000000000000000e+00; 0.000000000000000000e+00; 8.000000000000000000e+00}  ClassTemplateSpecKind=implicit  ClassTemplateParamNames={'NSamples'; 'ShiftAcc'; 'DiscardSample'; 'SwapRead'}  ClassTemplateParamKinds={'nontype'; 'nontype'; 'nontype'; 'nontype'}  ClassTemplateParamTypes={'int'; 'int'; 'bool'; 'bool'}  ClassTemplateParamValues={'512', '15', '1', '0'}  ClassCtorParamNames={'taps'}  ClassCtorParamSerializedTypes={'{R{Q1{C{Scint16}4}}}'}  ClassCtorParamValues={'[-160-111i 248+2878i 1183-239i -21-26i]'}  ClassIndex=1  ClassCtorIndex=1  ClassTabVisible=on  ClassTemplateParamsVisible=on  ClassCtorDeclVisible=on  ClassCtorParamsVisible=on  FunctionTabVisible=on  FunctionDecl=|  PortAttrs={ 'input', 'sin1', 'input_stream_cint16 * restrict', '', '', '', ''; 'input', 'sin2', 'input_stream_cint16 * restrict', '', '', '', ''; 'input', 'cin', 'input_stream< cacc48_t > *', '', '', '', ''; 'output', 'cout', 'output_stream< cacc48_t > *', '', '', '', 'OUTPUT_SIZE' }  PortAttrsEnables={'off', 'off', 'off', 'off', 'off', 'off', 'off';'off', 'off', 'off', 'off', 'off', 'off', 'off';'off', 'off', 'off', 'off', 'off', 'off', 'off';'off', 'off', 'off', 'off', 'off', 'off', 'on'}  SampleTime=-1  ClassDeclTypeOptions=|  ClassDecl=|  ClassTemplateParams={ 'NSamples', 'int', 'BURST_LENGTH'; 'ShiftAcc', 'int', 'SHIFT_ACC'; 'DiscardSample', 'bool', 'TRUE'; 'SwapRead', 'bool', 'FALSE' }  ClassTemplateParamsEnables={'off', 'off', 'on';'off', 'off', 'on';'off', 'off', 'on';'off', 'off', 'on'}  ClassCtorDeclTypeOptions=C[1 1]@t54@FIR_MultiKernel_cincout(cint16 const ( & taps ) [ 4 ])  ClassCtorDecl=FIR_MultiKernel_cincout(cint16 const ( & taps ) [ 4 ])  ClassCtorParams={ 'taps', 'cint16 const ( &) [ 4 ]', 'phi_5' }  KernelHeaderFile=FirDoubleStream.h  KernelClassName=DoubleStream::FIR_MultiKernel_cincout  KernelFunction=filter  KernelSourceFile=FirDoubleStream.cpp  KernelSearchPaths={'$SRC/aie_kernels'}  PreProcOptions={}  blockJsonConstraints="{\"type\":\"constraint\",\"constraintType\":\"location_kernel\",\"sid\":\"816\",\"lhs\":{\"type\":\"location\",\"templParam\":\"kernel\",\"args\":{\"type\":\"kernel\",\"name\":\"DualStreamSSR/SSR8/filter33\",\"sid\":\"816\"}},\"rhs\":{\"type\":\"tile\",\"args\":[{\"type\":\"evaluable\",\"expr\":\"24\",\"value\":24},{\"type\":\"evaluable\",\"expr\":\"4\",\"value\":4}]},\"equality\":true}"
      KernelAllAttrs=|
      | s[12;12;9;9;19;14;21;23;24;21;12;24;26;26;26;27;28;9;21;23;23;23;24;25;14;19;19;29]@FunctionNameDeclFileNamePortNamesPortTypesPortSerializedTypesPortDirectionsPortWindowSizeEnablesPortWindowMarginEnablesPortSynchronicityEnablesPortSignalSizeEnablesFunctionDeclFunctionTemplateSpecKindFunctionTemplateParamNamesFunctionTemplateParamKindsFunctionTemplateParamTypesFunctionTemplateParamValuesFunctionTemplateParamEnablesClassDeclClassTemplateSpecKindClassTemplateParamNamesClassTemplateParamKindsClassTemplateParamTypesClassTemplateParamValuesClassTemplateParamEnablesClassCtorDeclsClassCtorParamNamesClassCtorParamTypesClassCtorParamSerializedTypes[1 1]@C[28 1]@t6@filtert42@../../../aie/aie_kernels/FirDoubleStream.hC[4 1]@t4@sin1t4@sin2t3@cint4@coutC[4 1]@t30@input_stream_cint16 * restrictt30@input_stream_cint16 * restrictt26@input_stream< cacc48_t > *t27@output_stream< cacc48_t > *C[4 1]@t37@{Q2{P{Tinput_stream{1{t{Scint16}}}}}}t37@{Q2{P{Tinput_stream{1{t{Scint16}}}}}}t35@{P{Tinput_stream{1{t{Scacc48_t}}}}}t36@{P{Toutput_stream{1{t{Scacc48_t}}}}}C[4 1]@t5@inputt5@inputt5@inputt6@outputC[4 1]@l0@l0@l0@l0@C[4 1]@l0@l0@l0@l0@C[4 1]@l0@l0@l0@l0@C[4 1]@l0@l0@l0@l1@t281@namespace DoubleStream {
      | template < int NSamples, int ShiftAcc, bool DiscardSample, bool SwapRead > 
      | void FIR_MultiKernel_cincout::
      | filter(input_stream_cint16 * restrict sin1, input_stream_cint16 * restrict sin2, input_stream< cacc48_t > * cin, output_stream< cacc48_t > * cout);
      | }t4@nonee[0 1]@e[0 1]@e[0 1]@e[0 1]@e[0 1]@t132@namespace DoubleStream {
      | template < int NSamples, int ShiftAcc, bool DiscardSample, bool SwapRead > class FIR_MultiKernel_cincout;
      | }t8@implicitC[4 1]@t8@NSamplest8@ShiftAcct13@DiscardSamplet8@SwapReadC[4 1]@t7@nontypet7@nontypet7@nontypet7@nontypeC[4 1]@t3@intt3@intt4@boolt4@boolC[4 1]@nnnnC[4 1]@l1@l1@l1@l1@C[1 1]@t54@FIR_MultiKernel_cincout(cint16 const ( & taps ) [ 4 ])C[1 1]@C[1 1]@t4@tapsC[1 1]@C[1 1]@t23@cint16 const ( &) [ 4 ]C[1 1]@C[1 1]@t20@{R{Q1{C{Scint16}4}}}
      FunctionDecl=|
      | namespace DoubleStream {
      | template < int NSamples, int ShiftAcc, bool DiscardSample, bool SwapRead > 
      | void FIR_MultiKernel_cincout::
      | filter(input_stream_cint16 * restrict sin1, input_stream_cint16 * restrict sin2, input_stream< cacc48_t > * cin, output_stream< cacc48_t > * cout);
      | }
      ClassDeclTypeOptions=|
      | C[1 1]@t132@namespace DoubleStream {
      | template < int NSamples, int ShiftAcc, bool DiscardSample, bool SwapRead > class FIR_MultiKernel_cincout;
      | }
      ClassDecl=|
      | namespace DoubleStream {
      | template < int NSamples, int ShiftAcc, bool DiscardSample, bool SwapRead > class FIR_MultiKernel_cincout;
      | }
  filter34 : aieBasic/AIE Class Kernel  KernelAllAttrs=|  PortNames={'sin1'; 'sin2'; 'cin'; 'cout'}  PortSerializedTypes={'{Q2{P{Tinput_stream{1{t{Scint16}}}}}}'; '{Q2{P{Tinput_stream{1{t{Scint16}}}}}}'; '{P{Tinput_stream{1{t{Scacc48_t}}}}}'; '{P{Toutput_stream{1{t{Scacc48_t}}}}}'}  PortWindowSizes={0.000000000000000000e+00; 0.000000000000000000e+00; 0.000000000000000000e+00; 0.000000000000000000e+00}  PortWindowMargins={0.000000000000000000e+00; 0.000000000000000000e+00; 0.000000000000000000e+00; 0.000000000000000000e+00}  PortSynchronicities={'auto', 'auto', 'auto', 'auto'}  PortSignalSizes={0.000000000000000000e+00; 0.000000000000000000e+00; 0.000000000000000000e+00; 8.000000000000000000e+00}  ClassTemplateSpecKind=implicit  ClassTemplateParamNames={'NSamples'; 'ShiftAcc'; 'DiscardSample'; 'SwapRead'}  ClassTemplateParamKinds={'nontype'; 'nontype'; 'nontype'; 'nontype'}  ClassTemplateParamTypes={'int'; 'int'; 'bool'; 'bool'}  ClassTemplateParamValues={'512', '15', '1', '0'}  ClassCtorParamNames={'taps'}  ClassCtorParamSerializedTypes={'{R{Q1{C{Scint16}4}}}'}  ClassCtorParamValues={'[-160-111i 248+2878i 1183-239i -21-26i]'}  ClassIndex=1  ClassCtorIndex=1  ClassTabVisible=on  ClassTemplateParamsVisible=on  ClassCtorDeclVisible=on  ClassCtorParamsVisible=on  FunctionTabVisible=on  FunctionDecl=|  PortAttrs={ 'input', 'sin1', 'input_stream_cint16 * restrict', '', '', '', ''; 'input', 'sin2', 'input_stream_cint16 * restrict', '', '', '', ''; 'input', 'cin', 'input_stream< cacc48_t > *', '', '', '', ''; 'output', 'cout', 'output_stream< cacc48_t > *', '', '', '', 'OUTPUT_SIZE' }  PortAttrsEnables={'off', 'off', 'off', 'off', 'off', 'off', 'off';'off', 'off', 'off', 'off', 'off', 'off', 'off';'off', 'off', 'off', 'off', 'off', 'off', 'off';'off', 'off', 'off', 'off', 'off', 'off', 'on'}  SampleTime=-1  ClassDeclTypeOptions=|  ClassDecl=|  ClassTemplateParams={ 'NSamples', 'int', 'BURST_LENGTH'; 'ShiftAcc', 'int', 'SHIFT_ACC'; 'DiscardSample', 'bool', 'TRUE'; 'SwapRead', 'bool', 'FALSE' }  ClassTemplateParamsEnables={'off', 'off', 'on';'off', 'off', 'on';'off', 'off', 'on';'off', 'off', 'on'}  ClassCtorDeclTypeOptions=C[1 1]@t54@FIR_MultiKernel_cincout(cint16 const ( & taps ) [ 4 ])  ClassCtorDecl=FIR_MultiKernel_cincout(cint16 const ( & taps ) [ 4 ])  ClassCtorParams={ 'taps', 'cint16 const ( &) [ 4 ]', 'phi_5' }  KernelHeaderFile=FirDoubleStream.h  KernelClassName=DoubleStream::FIR_MultiKernel_cincout  KernelFunction=filter  KernelSourceFile=FirDoubleStream.cpp  KernelSearchPaths={'$SRC/aie_kernels'}  PreProcOptions={}  blockJsonConstraints="{\"type\":\"constraint\",\"constraintType\":\"location_kernel\",\"sid\":\"817\",\"lhs\":{\"type\":\"location\",\"templParam\":\"kernel\",\"args\":{\"type\":\"kernel\",\"name\":\"DualStreamSSR/SSR8/filter34\",\"sid\":\"817\"}},\"rhs\":{\"type\":\"tile\",\"args\":[{\"type\":\"evaluable\",\"expr\":\"25\",\"value\":25},{\"type\":\"evaluable\",\"expr\":\"5\",\"value\":5}]},\"equality\":true}"
      KernelAllAttrs=|
      | s[12;12;9;9;19;14;21;23;24;21;12;24;26;26;26;27;28;9;21;23;23;23;24;25;14;19;19;29]@FunctionNameDeclFileNamePortNamesPortTypesPortSerializedTypesPortDirectionsPortWindowSizeEnablesPortWindowMarginEnablesPortSynchronicityEnablesPortSignalSizeEnablesFunctionDeclFunctionTemplateSpecKindFunctionTemplateParamNamesFunctionTemplateParamKindsFunctionTemplateParamTypesFunctionTemplateParamValuesFunctionTemplateParamEnablesClassDeclClassTemplateSpecKindClassTemplateParamNamesClassTemplateParamKindsClassTemplateParamTypesClassTemplateParamValuesClassTemplateParamEnablesClassCtorDeclsClassCtorParamNamesClassCtorParamTypesClassCtorParamSerializedTypes[1 1]@C[28 1]@t6@filtert42@../../../aie/aie_kernels/FirDoubleStream.hC[4 1]@t4@sin1t4@sin2t3@cint4@coutC[4 1]@t30@input_stream_cint16 * restrictt30@input_stream_cint16 * restrictt26@input_stream< cacc48_t > *t27@output_stream< cacc48_t > *C[4 1]@t37@{Q2{P{Tinput_stream{1{t{Scint16}}}}}}t37@{Q2{P{Tinput_stream{1{t{Scint16}}}}}}t35@{P{Tinput_stream{1{t{Scacc48_t}}}}}t36@{P{Toutput_stream{1{t{Scacc48_t}}}}}C[4 1]@t5@inputt5@inputt5@inputt6@outputC[4 1]@l0@l0@l0@l0@C[4 1]@l0@l0@l0@l0@C[4 1]@l0@l0@l0@l0@C[4 1]@l0@l0@l0@l1@t281@namespace DoubleStream {
      | template < int NSamples, int ShiftAcc, bool DiscardSample, bool SwapRead > 
      | void FIR_MultiKernel_cincout::
      | filter(input_stream_cint16 * restrict sin1, input_stream_cint16 * restrict sin2, input_stream< cacc48_t > * cin, output_stream< cacc48_t > * cout);
      | }t4@nonee[0 1]@e[0 1]@e[0 1]@e[0 1]@e[0 1]@t132@namespace DoubleStream {
      | template < int NSamples, int ShiftAcc, bool DiscardSample, bool SwapRead > class FIR_MultiKernel_cincout;
      | }t8@implicitC[4 1]@t8@NSamplest8@ShiftAcct13@DiscardSamplet8@SwapReadC[4 1]@t7@nontypet7@nontypet7@nontypet7@nontypeC[4 1]@t3@intt3@intt4@boolt4@boolC[4 1]@nnnnC[4 1]@l1@l1@l1@l1@C[1 1]@t54@FIR_MultiKernel_cincout(cint16 const ( & taps ) [ 4 ])C[1 1]@C[1 1]@t4@tapsC[1 1]@C[1 1]@t23@cint16 const ( &) [ 4 ]C[1 1]@C[1 1]@t20@{R{Q1{C{Scint16}4}}}
      FunctionDecl=|
      | namespace DoubleStream {
      | template < int NSamples, int ShiftAcc, bool DiscardSample, bool SwapRead > 
      | void FIR_MultiKernel_cincout::
      | filter(input_stream_cint16 * restrict sin1, input_stream_cint16 * restrict sin2, input_stream< cacc48_t > * cin, output_stream< cacc48_t > * cout);
      | }
      ClassDeclTypeOptions=|
      | C[1 1]@t132@namespace DoubleStream {
      | template < int NSamples, int ShiftAcc, bool DiscardSample, bool SwapRead > class FIR_MultiKernel_cincout;
      | }
      ClassDecl=|
      | namespace DoubleStream {
      | template < int NSamples, int ShiftAcc, bool DiscardSample, bool SwapRead > class FIR_MultiKernel_cincout;
      | }
  filter35 : aieBasic/AIE Class Kernel  KernelAllAttrs=|  PortNames={'sin1'; 'sin2'; 'cin'; 'cout'}  PortSerializedTypes={'{Q2{P{Tinput_stream{1{t{Scint16}}}}}}'; '{Q2{P{Tinput_stream{1{t{Scint16}}}}}}'; '{P{Tinput_stream{1{t{Scacc48_t}}}}}'; '{P{Toutput_stream{1{t{Scacc48_t}}}}}'}  PortWindowSizes={0.000000000000000000e+00; 0.000000000000000000e+00; 0.000000000000000000e+00; 0.000000000000000000e+00}  PortWindowMargins={0.000000000000000000e+00; 0.000000000000000000e+00; 0.000000000000000000e+00; 0.000000000000000000e+00}  PortSynchronicities={'auto', 'auto', 'auto', 'auto'}  PortSignalSizes={0.000000000000000000e+00; 0.000000000000000000e+00; 0.000000000000000000e+00; 8.000000000000000000e+00}  ClassTemplateSpecKind=implicit  ClassTemplateParamNames={'NSamples'; 'ShiftAcc'; 'DiscardSample'; 'SwapRead'}  ClassTemplateParamKinds={'nontype'; 'nontype'; 'nontype'; 'nontype'}  ClassTemplateParamTypes={'int'; 'int'; 'bool'; 'bool'}  ClassTemplateParamValues={'512', '15', '1', '0'}  ClassCtorParamNames={'taps'}  ClassCtorParamSerializedTypes={'{R{Q1{C{Scint16}4}}}'}  ClassCtorParamValues={'[146-91i 4086+5221i 237-54i -83-21i]'}  ClassIndex=1  ClassCtorIndex=1  ClassTabVisible=on  ClassTemplateParamsVisible=on  ClassCtorDeclVisible=on  ClassCtorParamsVisible=on  FunctionTabVisible=on  FunctionDecl=|  PortAttrs={ 'input', 'sin1', 'input_stream_cint16 * restrict', '', '', '', ''; 'input', 'sin2', 'input_stream_cint16 * restrict', '', '', '', ''; 'input', 'cin', 'input_stream< cacc48_t > *', '', '', '', ''; 'output', 'cout', 'output_stream< cacc48_t > *', '', '', '', 'OUTPUT_SIZE' }  PortAttrsEnables={'off', 'off', 'off', 'off', 'off', 'off', 'off';'off', 'off', 'off', 'off', 'off', 'off', 'off';'off', 'off', 'off', 'off', 'off', 'off', 'off';'off', 'off', 'off', 'off', 'off', 'off', 'on'}  SampleTime=-1  ClassDeclTypeOptions=|  ClassDecl=|  ClassTemplateParams={ 'NSamples', 'int', 'BURST_LENGTH'; 'ShiftAcc', 'int', 'SHIFT_ACC'; 'DiscardSample', 'bool', 'TRUE'; 'SwapRead', 'bool', 'FALSE' }  ClassTemplateParamsEnables={'off', 'off', 'on';'off', 'off', 'on';'off', 'off', 'on';'off', 'off', 'on'}  ClassCtorDeclTypeOptions=C[1 1]@t54@FIR_MultiKernel_cincout(cint16 const ( & taps ) [ 4 ])  ClassCtorDecl=FIR_MultiKernel_cincout(cint16 const ( & taps ) [ 4 ])  ClassCtorParams={ 'taps', 'cint16 const ( &) [ 4 ]', 'phi_6' }  KernelHeaderFile=FirDoubleStream.h  KernelClassName=DoubleStream::FIR_MultiKernel_cincout  KernelFunction=filter  KernelSourceFile=FirDoubleStream.cpp  KernelSearchPaths={'$SRC/aie_kernels'}  PreProcOptions={}  blockJsonConstraints="{\"type\":\"constraint\",\"constraintType\":\"location_kernel\",\"sid\":\"818\",\"lhs\":{\"type\":\"location\",\"templParam\":\"kernel\",\"args\":{\"type\":\"kernel\",\"name\":\"DualStreamSSR/SSR8/filter35\",\"sid\":\"818\"}},\"rhs\":{\"type\":\"tile\",\"args\":[{\"type\":\"evaluable\",\"expr\":\"26\",\"value\":26},{\"type\":\"evaluable\",\"expr\":\"5\",\"value\":5}]},\"equality\":true}"
      KernelAllAttrs=|
      | s[12;12;9;9;19;14;21;23;24;21;12;24;26;26;26;27;28;9;21;23;23;23;24;25;14;19;19;29]@FunctionNameDeclFileNamePortNamesPortTypesPortSerializedTypesPortDirectionsPortWindowSizeEnablesPortWindowMarginEnablesPortSynchronicityEnablesPortSignalSizeEnablesFunctionDeclFunctionTemplateSpecKindFunctionTemplateParamNamesFunctionTemplateParamKindsFunctionTemplateParamTypesFunctionTemplateParamValuesFunctionTemplateParamEnablesClassDeclClassTemplateSpecKindClassTemplateParamNamesClassTemplateParamKindsClassTemplateParamTypesClassTemplateParamValuesClassTemplateParamEnablesClassCtorDeclsClassCtorParamNamesClassCtorParamTypesClassCtorParamSerializedTypes[1 1]@C[28 1]@t6@filtert42@../../../aie/aie_kernels/FirDoubleStream.hC[4 1]@t4@sin1t4@sin2t3@cint4@coutC[4 1]@t30@input_stream_cint16 * restrictt30@input_stream_cint16 * restrictt26@input_stream< cacc48_t > *t27@output_stream< cacc48_t > *C[4 1]@t37@{Q2{P{Tinput_stream{1{t{Scint16}}}}}}t37@{Q2{P{Tinput_stream{1{t{Scint16}}}}}}t35@{P{Tinput_stream{1{t{Scacc48_t}}}}}t36@{P{Toutput_stream{1{t{Scacc48_t}}}}}C[4 1]@t5@inputt5@inputt5@inputt6@outputC[4 1]@l0@l0@l0@l0@C[4 1]@l0@l0@l0@l0@C[4 1]@l0@l0@l0@l0@C[4 1]@l0@l0@l0@l1@t281@namespace DoubleStream {
      | template < int NSamples, int ShiftAcc, bool DiscardSample, bool SwapRead > 
      | void FIR_MultiKernel_cincout::
      | filter(input_stream_cint16 * restrict sin1, input_stream_cint16 * restrict sin2, input_stream< cacc48_t > * cin, output_stream< cacc48_t > * cout);
      | }t4@nonee[0 1]@e[0 1]@e[0 1]@e[0 1]@e[0 1]@t132@namespace DoubleStream {
      | template < int NSamples, int ShiftAcc, bool DiscardSample, bool SwapRead > class FIR_MultiKernel_cincout;
      | }t8@implicitC[4 1]@t8@NSamplest8@ShiftAcct13@DiscardSamplet8@SwapReadC[4 1]@t7@nontypet7@nontypet7@nontypet7@nontypeC[4 1]@t3@intt3@intt4@boolt4@boolC[4 1]@nnnnC[4 1]@l1@l1@l1@l1@C[1 1]@t54@FIR_MultiKernel_cincout(cint16 const ( & taps ) [ 4 ])C[1 1]@C[1 1]@t4@tapsC[1 1]@C[1 1]@t23@cint16 const ( &) [ 4 ]C[1 1]@C[1 1]@t20@{R{Q1{C{Scint16}4}}}
      FunctionDecl=|
      | namespace DoubleStream {
      | template < int NSamples, int ShiftAcc, bool DiscardSample, bool SwapRead > 
      | void FIR_MultiKernel_cincout::
      | filter(input_stream_cint16 * restrict sin1, input_stream_cint16 * restrict sin2, input_stream< cacc48_t > * cin, output_stream< cacc48_t > * cout);
      | }
      ClassDeclTypeOptions=|
      | C[1 1]@t132@namespace DoubleStream {
      | template < int NSamples, int ShiftAcc, bool DiscardSample, bool SwapRead > class FIR_MultiKernel_cincout;
      | }
      ClassDecl=|
      | namespace DoubleStream {
      | template < int NSamples, int ShiftAcc, bool DiscardSample, bool SwapRead > class FIR_MultiKernel_cincout;
      | }
  filter36 : aieBasic/AIE Class Kernel  KernelAllAttrs=|  PortNames={'sin1'; 'sin2'; 'cin'; 'cout'}  PortSerializedTypes={'{Q2{P{Tinput_stream{1{t{Scint16}}}}}}'; '{Q2{P{Tinput_stream{1{t{Scint16}}}}}}'; '{P{Tinput_stream{1{t{Scacc48_t}}}}}'; '{P{Toutput_stream{1{t{Scacc48_t}}}}}'}  PortWindowSizes={0.000000000000000000e+00; 0.000000000000000000e+00; 0.000000000000000000e+00; 0.000000000000000000e+00}  PortWindowMargins={0.000000000000000000e+00; 0.000000000000000000e+00; 0.000000000000000000e+00; 0.000000000000000000e+00}  PortSynchronicities={'auto', 'auto', 'auto', 'auto'}  PortSignalSizes={0.000000000000000000e+00; 0.000000000000000000e+00; 0.000000000000000000e+00; 8.000000000000000000e+00}  ClassTemplateSpecKind=implicit  ClassTemplateParamNames={'NSamples'; 'ShiftAcc'; 'DiscardSample'; 'SwapRead'}  ClassTemplateParamKinds={'nontype'; 'nontype'; 'nontype'; 'nontype'}  ClassTemplateParamTypes={'int'; 'int'; 'bool'; 'bool'}  ClassTemplateParamValues={'512', '15', '1', '0'}  ClassCtorParamNames={'taps'}  ClassCtorParamSerializedTypes={'{R{Q1{C{Scint16}4}}}'}  ClassCtorParamValues={'[342-439i 8773+2748i 102+525i -54+21i]'}  ClassIndex=1  ClassCtorIndex=1  ClassTabVisible=on  ClassTemplateParamsVisible=on  ClassCtorDeclVisible=on  ClassCtorParamsVisible=on  FunctionTabVisible=on  FunctionDecl=|  PortAttrs={ 'input', 'sin1', 'input_stream_cint16 * restrict', '', '', '', ''; 'input', 'sin2', 'input_stream_cint16 * restrict', '', '', '', ''; 'input', 'cin', 'input_stream< cacc48_t > *', '', '', '', ''; 'output', 'cout', 'output_stream< cacc48_t > *', '', '', '', 'OUTPUT_SIZE' }  PortAttrsEnables={'off', 'off', 'off', 'off', 'off', 'off', 'off';'off', 'off', 'off', 'off', 'off', 'off', 'off';'off', 'off', 'off', 'off', 'off', 'off', 'off';'off', 'off', 'off', 'off', 'off', 'off', 'on'}  SampleTime=-1  ClassDeclTypeOptions=|  ClassDecl=|  ClassTemplateParams={ 'NSamples', 'int', 'BURST_LENGTH'; 'ShiftAcc', 'int', 'SHIFT_ACC'; 'DiscardSample', 'bool', 'TRUE'; 'SwapRead', 'bool', 'FALSE' }  ClassTemplateParamsEnables={'off', 'off', 'on';'off', 'off', 'on';'off', 'off', 'on';'off', 'off', 'on'}  ClassCtorDeclTypeOptions=C[1 1]@t54@FIR_MultiKernel_cincout(cint16 const ( & taps ) [ 4 ])  ClassCtorDecl=FIR_MultiKernel_cincout(cint16 const ( & taps ) [ 4 ])  ClassCtorParams={ 'taps', 'cint16 const ( &) [ 4 ]', 'phi_7' }  KernelHeaderFile=FirDoubleStream.h  KernelClassName=DoubleStream::FIR_MultiKernel_cincout  KernelFunction=filter  KernelSourceFile=FirDoubleStream.cpp  KernelSearchPaths={'$SRC/aie_kernels'}  PreProcOptions={}  blockJsonConstraints="{\"type\":\"constraint\",\"constraintType\":\"location_kernel\",\"sid\":\"819\",\"lhs\":{\"type\":\"location\",\"templParam\":\"kernel\",\"args\":{\"type\":\"kernel\",\"name\":\"DualStreamSSR/SSR8/filter36\",\"sid\":\"819\"}},\"rhs\":{\"type\":\"tile\",\"args\":[{\"type\":\"evaluable\",\"expr\":\"27\",\"value\":27},{\"type\":\"evaluable\",\"expr\":\"5\",\"value\":5}]},\"equality\":true}"
      KernelAllAttrs=|
      | s[12;12;9;9;19;14;21;23;24;21;12;24;26;26;26;27;28;9;21;23;23;23;24;25;14;19;19;29]@FunctionNameDeclFileNamePortNamesPortTypesPortSerializedTypesPortDirectionsPortWindowSizeEnablesPortWindowMarginEnablesPortSynchronicityEnablesPortSignalSizeEnablesFunctionDeclFunctionTemplateSpecKindFunctionTemplateParamNamesFunctionTemplateParamKindsFunctionTemplateParamTypesFunctionTemplateParamValuesFunctionTemplateParamEnablesClassDeclClassTemplateSpecKindClassTemplateParamNamesClassTemplateParamKindsClassTemplateParamTypesClassTemplateParamValuesClassTemplateParamEnablesClassCtorDeclsClassCtorParamNamesClassCtorParamTypesClassCtorParamSerializedTypes[1 1]@C[28 1]@t6@filtert42@../../../aie/aie_kernels/FirDoubleStream.hC[4 1]@t4@sin1t4@sin2t3@cint4@coutC[4 1]@t30@input_stream_cint16 * restrictt30@input_stream_cint16 * restrictt26@input_stream< cacc48_t > *t27@output_stream< cacc48_t > *C[4 1]@t37@{Q2{P{Tinput_stream{1{t{Scint16}}}}}}t37@{Q2{P{Tinput_stream{1{t{Scint16}}}}}}t35@{P{Tinput_stream{1{t{Scacc48_t}}}}}t36@{P{Toutput_stream{1{t{Scacc48_t}}}}}C[4 1]@t5@inputt5@inputt5@inputt6@outputC[4 1]@l0@l0@l0@l0@C[4 1]@l0@l0@l0@l0@C[4 1]@l0@l0@l0@l0@C[4 1]@l0@l0@l0@l1@t281@namespace DoubleStream {
      | template < int NSamples, int ShiftAcc, bool DiscardSample, bool SwapRead > 
      | void FIR_MultiKernel_cincout::
      | filter(input_stream_cint16 * restrict sin1, input_stream_cint16 * restrict sin2, input_stream< cacc48_t > * cin, output_stream< cacc48_t > * cout);
      | }t4@nonee[0 1]@e[0 1]@e[0 1]@e[0 1]@e[0 1]@t132@namespace DoubleStream {
      | template < int NSamples, int ShiftAcc, bool DiscardSample, bool SwapRead > class FIR_MultiKernel_cincout;
      | }t8@implicitC[4 1]@t8@NSamplest8@ShiftAcct13@DiscardSamplet8@SwapReadC[4 1]@t7@nontypet7@nontypet7@nontypet7@nontypeC[4 1]@t3@intt3@intt4@boolt4@boolC[4 1]@nnnnC[4 1]@l1@l1@l1@l1@C[1 1]@t54@FIR_MultiKernel_cincout(cint16 const ( & taps ) [ 4 ])C[1 1]@C[1 1]@t4@tapsC[1 1]@C[1 1]@t23@cint16 const ( &) [ 4 ]C[1 1]@C[1 1]@t20@{R{Q1{C{Scint16}4}}}
      FunctionDecl=|
      | namespace DoubleStream {
      | template < int NSamples, int ShiftAcc, bool DiscardSample, bool SwapRead > 
      | void FIR_MultiKernel_cincout::
      | filter(input_stream_cint16 * restrict sin1, input_stream_cint16 * restrict sin2, input_stream< cacc48_t > * cin, output_stream< cacc48_t > * cout);
      | }
      ClassDeclTypeOptions=|
      | C[1 1]@t132@namespace DoubleStream {
      | template < int NSamples, int ShiftAcc, bool DiscardSample, bool SwapRead > class FIR_MultiKernel_cincout;
      | }
      ClassDecl=|
      | namespace DoubleStream {
      | template < int NSamples, int ShiftAcc, bool DiscardSample, bool SwapRead > class FIR_MultiKernel_cincout;
      | }
  filter37 : aieBasic/AIE Class Kernel  KernelAllAttrs=|  PortNames={'sin1'; 'sin2'; 'cin'; 'cout'}  PortSerializedTypes={'{Q2{P{Tinput_stream{1{t{Scint16}}}}}}'; '{Q2{P{Tinput_stream{1{t{Scint16}}}}}}'; '{P{Tinput_stream{1{t{Scacc48_t}}}}}'; '{P{Toutput_stream{1{t{Scacc48_t}}}}}'}  PortWindowSizes={0.000000000000000000e+00; 0.000000000000000000e+00; 0.000000000000000000e+00; 0.000000000000000000e+00}  PortWindowMargins={0.000000000000000000e+00; 0.000000000000000000e+00; 0.000000000000000000e+00; 0.000000000000000000e+00}  PortSynchronicities={'auto', 'auto', 'auto', 'auto'}  PortSignalSizes={0.000000000000000000e+00; 0.000000000000000000e+00; 0.000000000000000000e+00; 8.000000000000000000e+00}  ClassTemplateSpecKind=implicit  ClassTemplateParamNames={'NSamples'; 'ShiftAcc'; 'DiscardSample'; 'SwapRead'}  ClassTemplateParamKinds={'nontype'; 'nontype'; 'nontype'; 'nontype'}  ClassTemplateParamTypes={'int'; 'int'; 'bool'; 'bool'}  ClassTemplateParamValues={'512', '15', '0', '0'}  ClassCtorParamNames={'taps'}  ClassCtorParamSerializedTypes={'{R{Q1{C{Scint16}4}}}'}  ClassCtorParamValues={'[-54-21i 102-525i 8773-2748i 342+439i]'}  ClassIndex=1  ClassCtorIndex=1  ClassTabVisible=on  ClassTemplateParamsVisible=on  ClassCtorDeclVisible=on  ClassCtorParamsVisible=on  FunctionTabVisible=on  FunctionDecl=|  PortAttrs={ 'input', 'sin1', 'input_stream_cint16 * restrict', '', '', '', ''; 'input', 'sin2', 'input_stream_cint16 * restrict', '', '', '', ''; 'input', 'cin', 'input_stream< cacc48_t > *', '', '', '', ''; 'output', 'cout', 'output_stream< cacc48_t > *', '', '', '', 'OUTPUT_SIZE' }  PortAttrsEnables={'off', 'off', 'off', 'off', 'off', 'off', 'off';'off', 'off', 'off', 'off', 'off', 'off', 'off';'off', 'off', 'off', 'off', 'off', 'off', 'off';'off', 'off', 'off', 'off', 'off', 'off', 'on'}  SampleTime=-1  ClassDeclTypeOptions=|  ClassDecl=|  ClassTemplateParams={ 'NSamples', 'int', 'BURST_LENGTH'; 'ShiftAcc', 'int', 'SHIFT_ACC'; 'DiscardSample', 'bool', 'FALSE'; 'SwapRead', 'bool', 'FALSE' }  ClassTemplateParamsEnables={'off', 'off', 'on';'off', 'off', 'on';'off', 'off', 'on';'off', 'off', 'on'}  ClassCtorDeclTypeOptions=C[1 1]@t54@FIR_MultiKernel_cincout(cint16 const ( & taps ) [ 4 ])  ClassCtorDecl=FIR_MultiKernel_cincout(cint16 const ( & taps ) [ 4 ])  ClassCtorParams={ 'taps', 'cint16 const ( &) [ 4 ]', 'phi_0' }  KernelHeaderFile=FirDoubleStream.h  KernelClassName=DoubleStream::FIR_MultiKernel_cincout  KernelFunction=filter  KernelSourceFile=FirDoubleStream.cpp  KernelSearchPaths={'$SRC/aie_kernels'}  PreProcOptions={}  blockJsonConstraints="{\"type\":\"constraint\",\"constraintType\":\"location_kernel\",\"sid\":\"820\",\"lhs\":{\"type\":\"location\",\"templParam\":\"kernel\",\"args\":{\"type\":\"kernel\",\"name\":\"DualStreamSSR/SSR8/filter37\",\"sid\":\"820\"}},\"rhs\":{\"type\":\"tile\",\"args\":[{\"type\":\"evaluable\",\"expr\":\"28\",\"value\":28},{\"type\":\"evaluable\",\"expr\":\"5\",\"value\":5}]},\"equality\":true}"
